simulink library "etherlab_lib"  (Simulink 7.4)
settings: Solver=ode45  SolverMode=SingleTasking  StartTime=0.0  StopTime=10.0  RelTol=1e-3
undefined symbols (not defined in the file or in its folder): baumer_ecatencoder, ekxxxx, el1xxx, el2xxx, el320x_1, el331x, el3356, el3403, el37x2, el4xxx, el500x, el5021, El5152, EL51x1, el51xx, el9xxx, ep1xxx, ep2xxx, ep41xx_1, ep8309, murr_dio
(part 2 of 4)

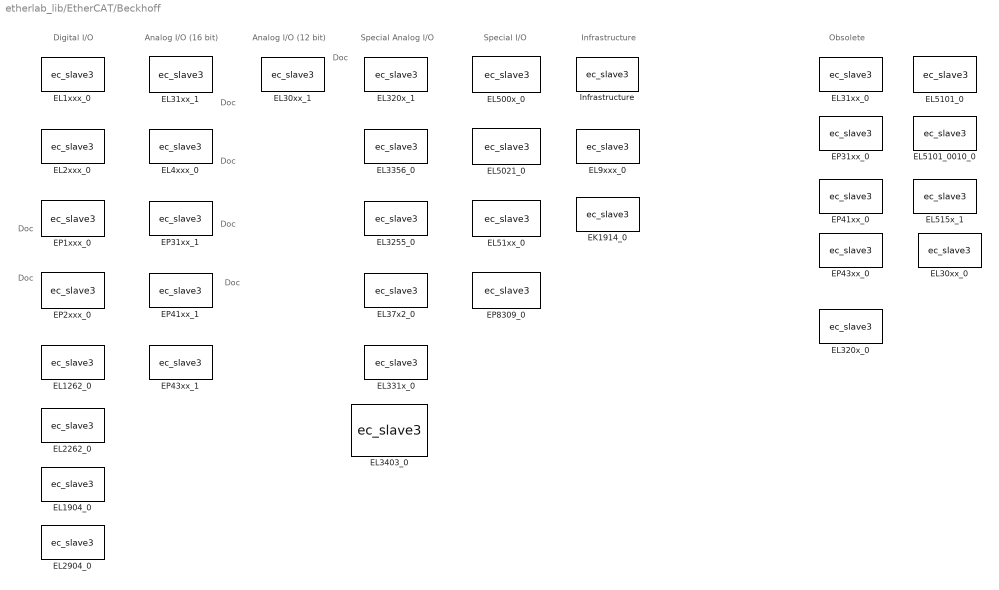
== system etherlab_lib/EtherCAT/Beckhoff ==
  note: Analog I/O (16 bit)
  note: Digital I/O
  note: Analog I/O (12 bit)
  note: Special Analog I/O
  note: Special I/O
  note: Infrastructure
  note: Obsolete
  note: Doc
  note: Doc
  note: Doc
  note: Doc
  note: Doc
  note: Doc
  note: Doc
  EK1914_0 : S-Function  FunctionName=ec_slave3  Parameters=Address,rv.SlaveConfig,rv.PortConfig,debug,tsample  SFunctionModules='ecrt_support'  EnableBusSupport=off  mask(EK1904){master=0, index=1, model=EK1914, stdio=on, safeio=off, tsample=-1, revision=, debug=}
      mask prompts: index "Slave Index"; model "Device Model"; stdio "Standard IO"; safeio "Safe IO"; tsample "Sample Time (-1 for inherited)"
      mask help: Beckhoff EtherCAT SAFE digital input/output coupler
      mask init:
      | Address = EtherCATSlave.formatAddress(master,index,tsample);
      | 
      | rv = ek1914(stdio, safeio);
      | 
      | text = sprintf('%s\\nM:%i Idx:%s', model, master, mat2str(index));
      | if numel(rv.PortConfig.input) > 1 || numel(rv.PortConfig.output) > 1
      |     EtherCATSlave.setPortNames(...
      |         {rv.PortConfig.input.portname},...
      |         {rv.PortConfig.output.portname});
      | 
      |     set_param(gcbh,'AttributesFormatString',text);
      | else
      |     set_param(gcbh,'AttributesFormatString','');
      |     set_param(gcbh,'MaskDisplay', strcat('disp(''',text,''')'));
      | end
      settings: AttributesFormatString=EK1914\nM:0 Idx:1
      mask Help: web(etherlab_help_path('ek1914.html'), '-helpbrowser');
      mask StyleString: edit,edit,popup(EK1914),checkbox,checkbox,edit,edit,edit
      mask Display:
      | port_label('input', 1, 'FSoE')
      | port_label('input', 2, 'StdOut')
      | port_label('output', 1, 'FSoE')
      | port_label('output', 2, 'StdIn')
  EL1262_0 : S-Function  FunctionName=ec_slave3  Parameters=Address,rv.SlaveConfig,rv.PortConfig,debug,tsample  SFunctionModules='ecrt_support'  EnableBusSupport=off  mask(EL1262){master=0, index=1, model=EL1262, one_ch=on, tsample=0, debug=0, revision=, dc_mode=10, dc_assign_activate=hex2dec('730'), dc_cycle0=0, dc_cycle0_factor=-10, dc_shift0=-10000, dc_shift0_factor=1, dc_shift0_input=off, dc_cycle1=0, dc_cycle1_factor=-1, dc_shift1=0, dc_shift1_factor=0}
      mask prompts: index "Slave Index"; model "Device Model"; one_ch "1 Ch. only"; tsample "Sample Time"; dc_mode "Mode/Oversampling"; dc_assign_activate "Assign Activate"; dc_cycle0 "Cycle Time Sync 0 [ns]"; dc_cycle0_factor "Factor"; dc_shift0 "Shift Time Sync0 [ns]"; dc_shift0_factor "Factor"; dc_shift0_input "Shift Time0 Input"; dc_cycle1 "Cycle Time Sync1 [ns]"; dc_cycle1_factor "Factor"; dc_shift1 "Shift Time Sync1 [ns]"; dc_shift1_factor "Factor"
      mask help: Beckhoff oversampling digital input
      mask init:
      | Address = EtherCATSlave.formatAddress(master,index,tsample);
      | 
      | rv = el1262(model).configure(one_ch,...
      |     [dc_mode, dc_assign_activate, ...
      |     dc_cycle0, dc_cycle0_factor,...
      |     dc_shift0, dc_shift0_factor, dc_shift0_input,...
      |     dc_cycle1, dc_cycle1_factor,...
      |     dc_shift1, dc_shift1_factor]);
      mask Help: web(etherlab_help_path('el1262.html'), '-helpbrowser');
      mask StyleString: edit,edit,popup(EL1262|EL1262-0050),checkbox,edit,edit,edit,popup(1|2|3|4|5|8|10|16|20|25|32|40|50|100|200|400|1000|Custom),edit,min,max,min,max,checkbox,min,max,min,max
      mask CallbackString: ||el1262().updateRevision()|||||EtherCATSlave.updateCustomDCEnable();||||||||||
      mask TabNameString: Main,Main,Main,Main,Main,Main,Main,Oversampling/DC,Oversampling/DC,Oversampling/DC,Oversampling/DC,Oversampling/DC,Oversampling/DC,Oversampling/DC,Oversampling/DC,Oversampling/DC,Oversampling/DC,Oversampling/DC
      mask Display: fprintf('%s\nM:%i Idx:%s', model, master, mat2str(index))
  EL1904_0 : S-Function  FunctionName=ec_slave3  Parameters=Address,rv.SlaveConfig,rv.PortConfig,debug,tsample  SFunctionModules='ecrt_support'  EnableBusSupport=off  mask(EL1904){master=0, index=1, model=EL1904, safein=off, tsample=-1, revision=, debug=}
      mask prompts: index "Slave Index"; model "Device Model"; safein "Safe inputs"; tsample "Sample Time (-1 for inherited)"
      mask help: Beckhoff EtherCAT SAFE digital input
      mask init:
      | Address = EtherCATSlave.formatAddress(master,index,tsample);
      | 
      | rv = el1904(safein);
      mask Help: web(etherlab_help_path('el1904.html'), '-helpbrowser');
      mask StyleString: edit,edit,popup(EL1904),checkbox,edit,edit,edit
      mask Display: fprintf('%s\nM:%i Idx:%s', model, master, mat2str(index))
  EL1xxx_0 : S-Function  LoadFcn=el1xxx().checkModelName  FunctionName=ec_slave3  Parameters=Address,rv.SlaveConfig,rv.PortConfig,debug,tsample  SFunctionModules='ecrt_support'  EnableBusSupport=off  mask(EL1xxx){master=0, index=1, model=EL1004, revision=, vector=on, tsample=0, debug=0}
      mask prompts: index "Slave Index"; model "Device Model"; vector "Vector Outputs"; tsample "Sample Time"; debug "Debug Level"
      mask help: Beckhoff EtherCAT Digital Input
      mask init:
      | Address = EtherCATSlave.formatAddress(master,index,tsample);
      | 
      | rv = el1xxx(model).configure(vector);
      mask Help: web(etherlab_help_path('el1xxx.html'), '-helpbrowser');
      mask StyleString: edit,edit,popup(EL1002|EL1004|EL1004-0010|EL1008|EL1012|EL1014|EL1014-0010|EL1018|EL1024|EL1034|EL1084|EL1088|EL1094|EL1098|EL1104|EL1114|EL1124|EL1134|EL1144|EL1202|EL1702|EL1702-0020|EL1712|EL1712-0020|EL1722|EL1804|EL1808|EL1809|EL1814|EL1819|EL1862|EL1862-0010|EL1872|EL1889),edit,checkbox,edit,edit
      mask CallbackString: ||el1xxx().updateRevision()||||
      mask Display: fprintf('%s\nM:%i Idx:%s', model, master, mat2str(index))
  EL2262_0 : S-Function  FunctionName=ec_slave3  Parameters=Address,rv.SlaveConfig,rv.PortConfig,debug,tsample  SFunctionModules='ecrt_support'  EnableBusSupport=off  mask(EL2262){master=0, index=1, model=EL2262, one_ch=on, tsample=0, debug=0, revision=, dc_mode=10, dc_assign_activate=hex2dec('730'), dc_cycle0=0, dc_cycle0_factor=-10, dc_shift0=-10000, dc_shift0_factor=1, dc_shift0_input=off, dc_cycle1=0, dc_cycle1_factor=-1, dc_shift1=0, dc_shift1_factor=0}
      mask prompts: index "Slave Index"; model "Device Model"; one_ch "1 Ch. only"; tsample "Sample Time"; dc_mode "Mode/Oversampling"; dc_assign_activate "Assign Activate"; dc_cycle0 "Cycle Time Sync 0 [ns]"; dc_cycle0_factor "Factor"; dc_shift0 "Shift Time Sync0 [ns]"; dc_shift0_factor "Factor"; dc_shift0_input "Shift Time0 Input"; dc_cycle1 "Cycle Time Sync1 [ns]"; dc_cycle1_factor "Factor"; dc_shift1 "Shift Time Sync1 [ns]"; dc_shift1_factor "Factor"
      mask help: Beckhoff oversampling digital output
      mask init:
      | Address = EtherCATSlave.formatAddress(master,index,tsample);
      | 
      | rv = el2262(model).configure(one_ch,...
      |     [dc_mode, dc_assign_activate, ...
      |     dc_cycle0, dc_cycle0_factor,...
      |     dc_shift0, dc_shift0_factor, dc_shift0_input,...
      |     dc_cycle1, dc_cycle1_factor,...
      |     dc_shift1, dc_shift1_factor]);
      mask Help: web(etherlab_help_path('el2262.html'), '-helpbrowser');
      mask StyleString: edit,edit,popup(EL2262),checkbox,edit,edit,edit,popup(1|2|3|4|5|8|10|16|20|25|32|40|50|100|200|400|1000|Custom),edit,min,max,min,max,checkbox,min,max,min,max
      mask CallbackString: ||el2262().updateRevision()|||||EtherCATSlave.updateCustomDCEnable();||||||||||
      mask TabNameString: Main,Main,Main,Main,Main,Main,Main,Oversampling/DC,Oversampling/DC,Oversampling/DC,Oversampling/DC,Oversampling/DC,Oversampling/DC,Oversampling/DC,Oversampling/DC,Oversampling/DC,Oversampling/DC,Oversampling/DC
      mask Display: fprintf('%s\nM:%i Idx:%s', model, master, mat2str(index))
  EL2904_0 : S-Function  FunctionName=ec_slave3  Parameters=Address,rv.SlaveConfig,rv.PortConfig,debug,tsample  SFunctionModules='ecrt_support'  EnableBusSupport=off  mask(EL2904){master=0, index=1, model=EL2904, safeout=off, tsample=-1, revision=, debug=}
      mask prompts: index "Slave Index"; model "Device Model"; safeout "Safe outputs"; tsample "Sample Time (-1 for inherited)"
      mask help: Beckhoff EtherCAT SAFE digital output
      mask init:
      | Address = EtherCATSlave.formatAddress(master,index,tsample);
      | 
      | rv = el2904(safeout);
      mask Help: web(etherlab_help_path('el2904.html'), '-helpbrowser');
      mask StyleString: edit,edit,popup(EL2904),checkbox,edit,edit,edit
      mask Display: fprintf('%s\nM:%i Idx:%s', model, master, mat2str(index))
  EL2xxx_0 : S-Function  LoadFcn=el2xxx().checkModelName  FunctionName=ec_slave3  Parameters=Address,rv.SlaveConfig,rv.PortConfig,debug,tsample  SFunctionModules='ecrt_support'  EnableBusSupport=off  mask(EL2xxx){master=0, index=1, model=EL2004, revision=, vector=on, diag=off, tsample=-1, debug=0}
      mask prompts: index "Slave Index"; model "Device Model"; vector "Vector Inputs"; diag "Diag Port"; tsample "Sample Time (-1 for inherited)"
      mask help: Beckhoff EtherCAT Digital Output
      mask init:
      | Address = EtherCATSlave.formatAddress(master,index,tsample);
      | 
      | rv = el2xxx(model).configure(vector,diag);
      mask Help: web(etherlab_help_path('el2xxx.html'), '-helpbrowser')
      mask StyleString: edit,edit,popup(EL2002|EL2004|EL2008|EL2022|EL2024|EL2024-0010|EL2032|EL2034|EL2042|EL2084|EL2088|EL2124|EL2202|EL2202-0100|EL2602|EL2612|EL2622|EL2624|EL2652|EL2712|EL2722|EL2722-0010|EL2732|EL2784|EL2788|EL2794|EL2798|EL2808|EL2809|EL2828|EL2872|EL2872-0010|EL2889|EL2004-0000-0000|EL2032-0000-0000|EM2042),edit,checkbox,checkbox,edit,edit
      mask CallbackString: ||el2xxx().modelChanged()|||||
      mask Display: fprintf('%s\nM:%i Idx:%s', model, master, mat2str(index))
  EL30xx_0 : S-Function  LoadFcn=|  FunctionName=ec_slave3  Parameters=Address,rv.SlaveConfig,rv.PortConfig,debug,tsample  SFunctionModules='ecrt_support'  EnableBusSupport=off  mask(EL30xx){master=0, index=1, model=EL3002, vector=on, raw=off, scale=, offset=, tau=, tsample=0, debug=0}
      | el30xx('check')
      | if ~strcmp(bdroot(gcb),'etherlab_lib')
      |   disp([gcb ' is obsolete. Please replace'])
      | end
      mask prompts: index "Slave Index"; model "Device Model"; vector "Vector Output"; raw "Raw Bits"; scale "Output Scale"; offset "Output Offset"; tau "LPF Time Constant (sec)"; tsample "Sample Time"
      mask help: Beckhoff 1,2,4,8-Channel 16-Bit Analog Input
      mask init:
      | Address = EtherCATSlave.formatAddress(master,index,tsample);
      | 
      | el30xx('set');
      | 
      | rv = get_param(gcbh, 'UserData');
      mask StyleString: edit,edit,popup(EL3001|EL3002|EL3004|EL3008|EL3011|EL3012|EL3014|EL3021|EL3022|EL3024|EL3041|EL3042|EL3044|EL3048|EL3051|EL3052|EL3054|EL3058|EL3061|EL3062|EL3062-0030|EL3064|EL3068),checkbox,checkbox,edit,edit,edit,edit,edit
      mask CallbackString: ||el30xx('set');|el30xx('set');||||||
      mask Display:
      | fprintf('%s\n%s AIn\nM:%i Idx:%s', ...
      |     model, rv.SlaveConfig.function, master, mat2str(index))
  EL30xx_1 : S-Function  LoadFcn=|  FunctionName=ec_slave3  Parameters=Address,rv.SlaveConfig,rv.PortConfig,debug,tsample  SFunctionModules='ecrt_support'  EnableBusSupport=off  mask(EL30xx){master=0, index=1, model=EL3002, revision=, vector=on, status=off, gain=[], offset=[], tau=[], tsample=0, debug=0, omega=, filter=Off, opmode=FreeRun, fastop=off}
      | el30xx_1().checkModelName()
      | EtherCATSlave.checkFilter()
      mask prompts: index "Slave Index"; model "Device Model"; vector "Vector Output"; status "Status Output"; gain "Output Scale"; offset "Output Offset"; tau "LPF time constant (s)"; tsample "Sample Time"; omega "deprecated"; opmode "Synchronization Mode (1C33:01.0)"; fastop "FastOp Mode (1C33:01.15)"
      mask help: Beckhoff 1,2,4,8-Channel 16-Bit Analog Input
      mask init:
      | Address = EtherCATSlave.formatAddress(master,index,tsample);
      | 
      | rv = el30xx_1(model).configure(status,vector,...
      |     EtherCATSlave.configureScale(2^15,gain,offset,tau),...
      |     [filter,opmode,fastop]);
      | 
      | if vector
      |     set_param(gcb,'AttributesFormatString','');
      | 
      |     set_param(gcb,'MaskDisplay',...
      |         sprintf('disp(''%s %s\\nM:%i Idx:%s'')',...
      |         model,rv.function,master,mat2str(index)))
      | else
      |     EtherCATSlave.setPortNames({},...
      |         {rv.PortConfig.output.portname})
      |     
      |     set_param(gcb,'AttributesFormatString',...
      |         sprintf('%s %s\nM:%i Idx:%s',...
      |         model,rv.function,master,mat2str(index)))
      | end
      mask StyleString: edit,edit,popup(EL3001|EL3002|EL3004|EL3008|EL3011|EL3012|EL3014|EL3021|EL3022|EL3024|EL3041|EL3042|EL3042-0017|EL3044|EL3048|EL3051|EL3052|EL3054|EL3058|EL3061|EL3062|EL3062-0015|EL3062-0030|EL3064|EL3068|EL3001-0000-0018|EL3002-0000-0018|EL3004-0000-0018|EL3008-0000-0018|EL3011-0000-0016|EL3012-0000-0016|EL3014-0000-0016|EL3021-0000-0016|EL3022-0000-0016|EL3024-0000-0016|EL3041-0000-0017|EL3042-0000-0017|EL3044-0000-0017|EL3048-0000-0017|EL3051-0000-0017|EL3052-0000-0017|EL3054-0000-0017|EL3058-0000-0017|EL3061-0000-0017|EL3062-0000-0017|EL3062-0030-0017|EL3064-0000-0017|EL3068-0000-0017),edit,checkbox,checkbox,edit,edit,edit,edit,edit,edit,popup(Off|50Hz FIR|60Hz FIR|IIR 1|IIR 2|IIR 3|IIR 4|IIR 5|IIR 6|IIR 7|IIR 8),popup(FreeRun|FrameTriggered SM2),checkbox
      mask CallbackString: ||el30xx_1().updateRevision()||||||||||el30xx_1.updateFilter||
      mask TabNameString: Main,Main,Main,Main,Main,Main,Main,Main,Main,Main,Main,Main,Filter,Filter,Filter
      mask Display: disp('EL3002 +-10V\nM:0 Idx:1')
  EL31xx_0 : S-Function  LoadFcn=|  FunctionName=ec_slave3  Parameters=Address,rv.SlaveConfig,rv.PortConfig,debug,tsample  SFunctionModules='ecrt_support'  EnableBusSupport=off  mask(EL31xx){master=0, index=1, model=EL3102, dc=DC-Synchron, vector=on, raw=off, scale=, offset=, tau=, tsample=0, debug=0}
      | el31xx('check')
      | if ~strcmp(bdroot(gcb),'etherlab_lib')
      |   disp([gcb ' is obsolete. Please replace'])
      | end
      mask prompts: index "Slave Index"; model "Device Model"; dc "Distributed Clock"; vector "Vector Output"; raw "Raw output"; scale "Output Scale"; offset "Output Offset"; tau "LPF Time Constant (sec)"; tsample "Sample Time"
      mask help:
      | Beckhoff 2,4,8-Channel 16-Bit Analog Input with Distributed Clocks
      |
      | Status output is not supported
      mask init:
      | Address = EtherCATSlave.formatAddress(master,index,tsample);
      | 
      | el31xx('set');  % Report errors
      | 
      | rv = get_param(gcb,'UserData');
      mask Help:
      | This block generically implements the EtherCAT 16-Bit Analog Input Terminal for various models.
      | <p/>
      | The following Terminals are supported:
      | <center>
      | <table width="80%">
      | <tr><td>EL3102,4,8</td><td>-10..10V Voltage Input</td></tr>
      | <tr><td>EL3112,4   </td><td>0..20mA Current Input</td></tr>
      | <tr><td>EL3122,4   </td><td>4..20mA Current Input</td></tr>
      | <tr><td>EL3142,4,8</td><td>0..20mA Current Input</td></tr>
      | <tr><td>EL3152,4,8</td><td>4..20mA Current Input</td></tr>
      | <tr><td>EL3162,4,8</td><td>0..10V Voltage Input</td></tr>
      | </table>
      | </center>
      | <p/>
      | Choose and set the following options:
      | <h4>Master:</h4>
      | Set the EtherCAT Master of this terminal.
      | 
      | <h4>Slave Index:</h4>
      | Set the EtherCAT slave index. Following address formats are allowed:
      | <ol>
      | <li> Absolute addressing: a scalar number <<b><tt>n</tt></b>> representing the (zero based) absolute position in the bus.
      | <li> SSId addressing: the Secondary Slave (or 'Alias') Addressing has the form <<b><tt>[alias position]</tt></b>> where <b><tt>alias</tt></b> is the Secondary Slave Id of the EtherCAT slave and <b><tt>position</tt></b> is the offset after the slave with the given <b><tt>alias</tt></b>. The SSId has to be preprogrammed into the slave with other service tools (see 'ethercat alias --help').
      | </ol>
      | 
      | <h4>Device Model:</h4>
      | Choose the model at the Indexed position of the master.
      | 
      | <h4>Output Type:</h4>
      | <ul>
      | <li>Choose <b>Vector Output</b> to have a single output as a vector
      | with a size corresponding to the channel count of the terminal. This mode also allows a status output port to be displayed. <br/>
      | <li>Choose <b>Separate Outputs</b> to have one output for every channel.
      | </ul>
      | <h4>Output Full Scale</h4>
      | When <b>Output Data Type</b> is set to <b>Double with scale and offset</b>, the block's output value at full scale terminal input can be set here.
      | 
      | <h4>Output Offset</h4>
      | When <b>Output Data Type</b> is set to <b>Double with scale and offset</b>, the blocks output at zero terminal input can be set here. Note that the Full Scale above is also increased by this amount. Note furthermore that this corresponds to the minimum input for terminals such as 4..20mA.
      | 
      | <h4>Output Data Type</h4>
      | Choose the block's output data type for the output signal. Available are:
      | <ul>
      | <li><b><tt>Raw</tt></b> outputting the internal raw value as <tt>int16_T</tt> or <tt>uint16_T</tt> as appropriate
      | <li><b><tt>Double</tt></b> outputting 0..10, -10..10, 0..0.02 and 0.004..0.02 depending on the Model as appropriate
      | <li><b><tt>Double with scale and offset</tt></b>, allowing the output to be scaled with an offset.
      | </ul>
      | 
      | <p>
      | Choosing <b>Status Output</b> provides a port of type <tt>uint8_T</tt> where the status is presented. This is only enabled when <b>Vector Output</b> is selected. Terminal input over- and underrange can be detected using this output. See the terminal's documentation.
      | 
      | <h4>Output Filter</h4>
      | When not in <b>Raw</b> mode, the <b>Output Filter</b> checkbox becomes available, allowing the use of an internal low pass filter. Enter the <b>LPF Time Constant</b> for the filter in the field below.
      | <br>For continuous sample time systems (0 in Sample Time), the filter is also continuous. Discrete samples systems (Sample Time > 0) uses an equivalent discrete low pass filter with a similar time constant.
      | 
      | <p>
      | Set the <b>Sample Time</b> for the block. <tt>0</tt> is continuous sample time (runs at the model's base rate). Setting <tt>-1</tt> will try to set the time using back propagation.
      mask StyleString: edit,edit,popup(EL3101|EL3102|EL3104|EL3111|EL3112|EL3114|EL3121|EL3122|EL3124|EL3141|EL3142|EL3142-010|EL3144|EL3151|EL3152|EL3154|EL3161|EL3162|EL3164),popup(Free Run|DC-Synchron|DC-Synchron (input based)),checkbox,checkbox,edit,edit,edit,edit,edit
      mask CallbackString: ||el31xx('set')|el31xx('set')|el31xx('set')||||||
      mask Display:
      | fprintf('%s\n%s AIn\nM:%i Idx:%s', ...
      |     model, rv.SlaveConfig.function, master, mat2str(index))
  EL31xx_1 : S-Function  LoadFcn=|  FunctionName=ec_slave3  Parameters=Address,rv.SlaveConfig,rv.PortConfig,debug,tsample  SFunctionModules='ecrt_support'  EnableBusSupport=off  mask(EL31xx){master=0, index=1, model=EL3102, revision=, vector=on, status=off, filter=Off, gain=[], offset=[], tau=[], tsample=0, debug=0, omega=, dc_mode=Free Run/SM-Synchron, dc_assign_activate=hex2dec('700'), dc_cycle0=[], dc_cycle0_factor=[], dc_shift0=[], dc_shift0_factor=[], dc_shift0_input=off, dc_cycle1=[], dc_cycle1_factor=[], dc_shift1=[], dc_shift1_factor=[]}
      | el31xx_1().checkModelName()
      | EtherCATSlave.checkFilter()
      mask prompts: index "Slave Index"; model "Device Model"; vector "Vector Output"; status "Status output"; gain "Output Gain"; offset "Output Offset"; tau "LPF time constant (s)"; tsample "Sample Time"; omega "deprecated"; dc_mode "Mode"; dc_assign_activate "Assign Activate"; dc_cycle0 "Cycle Time Sync 0"; dc_cycle0_factor "Factor"; dc_shift0 "Shift Time Sync0"; dc_shift0_factor "Factor"; dc_shift0_input "Shift Time0 Input"; dc_cycle1 "Cycle Time Sync1"; dc_cycle1_factor "Factor"; dc_shift1 "Shift Time Sync1"; dc_shift1_factor "Factor"
      mask help: Beckhoff 2,4,8-Channel 16-Bit Analog Input with Distributed Clocks
      mask init:
      | Address = EtherCATSlave.formatAddress(master,index,tsample);
      | 
      | rv = el31xx_1(model).configure(status,vector,...
      |     EtherCATSlave.configureScale(2^15,gain,offset,tau),...
      |     [dc_mode, dc_assign_activate, ...
      |      dc_cycle0, dc_cycle0_factor, ...
      |      dc_shift0, dc_shift0_factor, dc_shift0_input, ...
      |      dc_cycle1, dc_cycle1_factor, ...
      |      dc_shift1, dc_shift1_factor], ...
      |      filter);
      |  
      | if vector || model(6) == '1'
      |     set_param(gcb,'AttributesFormatString','');
      | 
      |     set_param(gcb,'MaskDisplay',...
      |         sprintf('disp(''%s\\nM:%i Idx:%s'')',...
      |         model,master,mat2str(index)))
      | else
      |     EtherCATSlave.setPortNames({},...
      |         {rv.PortConfig.output.portname})
      |     
      |     set_param(gcb,'AttributesFormatString',...
      |         sprintf('%s\nM:%i Idx:%s',...
      |         model,master,mat2str(index)))
      | end
      mask Help:
      | This block generically implements the EtherCAT 16-Bit Analog Input Terminal for various models.
      | <p/>
      | The following Terminals are supported:
      | <center>
      | <table width="80%">
      | <tr><td>EL3102,4,8</td><td>-10..10V Voltage Input</td></tr>
      | <tr><td>EL3112,4   </td><td>0..20mA Current Input</td></tr>
      | <tr><td>EL3122,4   </td><td>4..20mA Current Input</td></tr>
      | <tr><td>EL3142,4,8</td><td>0..20mA Current Input</td></tr>
      | <tr><td>EL3152,4,8</td><td>4..20mA Current Input</td></tr>
      | <tr><td>EL3162,4,8</td><td>0..10V Voltage Input</td></tr>
      | </table>
      | </center>
      | <p/>
      | Choose and set the following options:
      | <h4>Master:</h4>
      | Set the EtherCAT Master of this terminal.
      | 
      | <h4>Slave Index:</h4>
      | Set the EtherCAT slave index. Following address formats are allowed:
      | <ol>
      | <li> Absolute addressing: a scalar number <<b><tt>n</tt></b>> representing the (zero based) absolute position in the bus.
      | <li> SSId addressing: the Secondary Slave (or 'Alias') Addressing has the form <<b><tt>[alias position]</tt></b>> where <b><tt>alias</tt></b> is the Secondary Slave Id of the EtherCAT slave and <b><tt>position</tt></b> is the offset after the slave with the given <b><tt>alias</tt></b>. The SSId has to be preprogrammed into the slave with other service tools (see 'ethercat alias --help').
      | </ol>
      | 
      | <h4>Device Model:</h4>
      | Choose the model at the Indexed position of the master.
      | 
      | <h4>Output Type:</h4>
      | <ul>
      | <li>Choose <b>Vector Output</b> to have a single output as a vector
      | with a size corresponding to the channel count of the terminal. This mode also allows a status output port to be displayed. <br/>
      | <li>Choose <b>Separate Outputs</b> to have one output for every channel.
      | </ul>
      | <h4>Output Full Scale</h4>
      | When <b>Output Data Type</b> is set to <b>Double with scale and offset</b>, the block's output value at full scale terminal input can be set here.
      | 
      | <h4>Output Offset</h4>
      | When <b>Output Data Type</b> is set to <b>Double with scale and offset</b>, the blocks output at zero terminal input can be set here. Note that the Full Scale above is also increased by this amount. Note furthermore that this corresponds to the minimum input for terminals such as 4..20mA.
      | 
      | <h4>Output Data Type</h4>
      | Choose the block's output data type for the output signal. Available are:
      | <ul>
      | <li><b><tt>Raw</tt></b> outputting the internal raw value as <tt>int16_T</tt> or <tt>uint16_T</tt> as appropriate
      | <li><b><tt>Double</tt></b> outputting 0..10, -10..10, 0..0.02 and 0.004..0.02 depending on the Model as appropriate
      | <li><b><tt>Double with scale and offset</tt></b>, allowing the output to be scaled with an offset.
      | </ul>
      | 
      | <p>
      | Choosing <b>Status Output</b> provides a port of type <tt>uint8_T</tt> where the status is presented. This is only enabled when <b>Vector Output</b> is selected. Terminal input over- and underrange can be detected using this output. See the terminal's documentation.
      | 
      | <h4>Output Filter</h4>
      | When not in <b>Raw</b> mode, the <b>Output Filter</b> checkbox becomes available, allowing the use of an internal low pass filter. Enter the <b>LPF Time Constant</b> for the filter in the field below.
      | <br>For continuous sample time systems (0 in Sample Time), the filter is also continuous. Discrete samples systems (Sample Time > 0) uses an equivalent discrete low pass filter with a similar time constant.
      | 
      | <p>
      | Set the <b>Sample Time</b> for the block. <tt>0</tt> is continuous sample time (runs at the model's base rate). Setting <tt>-1</tt> will try to set the time using back propagation.
      mask StyleString: edit,edit,popup(EL3101|EL3102|EL3104|EL3111|EL3112|EL3114|EL3121|EL3122|EL3124|EL3141|EL3142|EL3142-0010|EL3144|EL3151|EL3152|EL3154|EL3161|EL3162|EL3164|EL3101-0000-0016|EL3102-0000-0017|EL3104-0000-0016|EL3111-0000-0016|EL3112-0000-0017|EL3114-0000-0017|EL3121-0000-0016|EL3122-0000-0017|EL3124-0000-0016|EL3141-0000-0016|EL3142-0000-0017|EL3142-0010-0017|EL3144-0000-0016|EL3151-0000-0016|EL3152-0000-0017|EL3154-0000-0016|EL3161-0000-0016|EL3162-0000-0017|EL3164-0000-0016),edit,checkbox,checkbox,popup(Off|50Hz FIR|60Hz FIR|IIR 1|IIR 2|IIR 3|IIR 4|IIR 5|IIR 6|IIR 7|IIR 8),edit,edit,edit,edit,edit,edit,popup(Free Run/SM-Synchron|DC-Synchron|DC-Synchron (input based)|Custom),edit,min,max,min,max,checkbox,min,max,min,max
      mask CallbackString: ||el31xx_1().updateRevision()|el31xx_1().updateRevision()||||||||||EtherCATSlave.updateCustomDCEnable()||||||||||
      mask TabNameString: Main,Main,Main,Main,Main,Main,Main,Main,Main,Main,Main,Main,Main,Distributed Clocks,Distributed Clocks,Distributed Clocks,Distributed Clocks,Distributed Clocks,Distributed Clocks,Distributed Clocks,Distributed Clocks,Distributed Clocks,Distributed Clocks,Distributed Clocks
      mask Display: disp('EL3102\nM:0 Idx:1')
  EL320x_0 : S-Function  LoadFcn=|  FunctionName=ec_slave3  Parameters=Address,rv.SlaveConfig,rv.PortConfig,debug,tsample  SFunctionModules='ecrt_support'  EnableBusSupport=off  mask(EL320x){master=0, index=1, model=EL3204, rtd=0, technology=2, filter=50 Hz, vector=on, enable_status=on, tsample=0, debug=0}
      | el320x('check')
      | if ~strcmp(bdroot(gcb),'etherlab_lib')
      |   disp([gcb ' is obsolete. Please replace'])
      | end
      mask prompts: index "Slave Index"; model "Device Model"; rtd "RTD-Element (CoE 80x0:19)"; technology "Connection Technology (CoE 80x0:1A)"; filter "Filter (CoE 8000:15)"; vector "Vector Output"; enable_status "Status Port"; tsample "Sample Time"
      mask help: Beckhoff 1, 2, 4-Channel Input Terminal Pt100 (RTD)
      mask init:
      | Address = EtherCATSlave.formatAddress(master,index,tsample);
      | 
      | SdoConfig = [];
      | 
      | rv = get_param(gcbh,'UserData');
      | 
      | count = numel(rv.SlaveConfig.sm{1}{3});
      | 
      | err = {};
      | if numel(rtd) == 1
      |     rtd = repmat(rtd,1,count);
      | elseif numel(rtd) ~= count
      |     err = {['- Mask option "RTD Element"' ...
      |         ' is not a scalar or vector with ' ...
      |         num2str(count) ' elements']};
      | end
      | 
      | if numel(technology) == 1
      |     technology = repmat(technology,1,count);
      | elseif numel(technology) ~= count
      |     err = horzcat(err, ['- Mask option "Connection Technology"' ...
      |         ' is not a scalar or vector with ' ...
      |         num2str(count) ' elements']);
      | end
      | 
      | if ~isempty(err)
      |     errordlg(err,gcb);
      |     return
      | end
      | 
      | rv.SlaveConfig.sdo = num2cell(vertcat(...
      |     [hex2dec('8000'),6,8,1],...
      |     [hex2dec('8000'),hex2dec('15'),16,filter+1],...
      |     horzcat(repmat(hex2dec('8000') + 16*(0:count-1)',2,1),...
      |             [hex2dec('19')*ones(count,1);hex2dec('1a')*ones(count,1)],...
      |             16*ones(count*2,1),...
      |             vertcat(reshape(rtd,[],1),...
      |                     reshape(technology,[],1)))));
      mask Help: web(etherlab_help_path('el320x.html'), '-helpbrowser');
      mask StyleString: edit,edit,popup(EL3201|EL3201-0010|EL3201-0020|EL3202|EL3202-0010|EL3204),edit,edit,popup(50 Hz|60 Hz|100 Hz|500 Hz|1 kHz|2 kHz|3.75 kHz|7.5 kHz|15 kHz|30 kHz|5 Hz|10 Hz),checkbox,checkbox,edit,edit
      mask CallbackString: ||el320x('set');||||el320x('set');|el320x('set');||
      mask Display: fprintf('%s\nRTD In\n%i Idx:%s', model, master, mat2str(index))
  EL320x_1 : S-Function  LoadFcn=el320x_1().checkModelName()  FunctionName=ec_slave3  Parameters=Address,rv.SlaveConfig,rv.PortConfig,debug,tsample  SFunctionModules='ecrt_support'  EnableBusSupport=off  mask(EL320x){master=0, index=1, model=EL3201, revision=, filter=Off, vector=on, status=off, tsample=0, debug=0, sdo_01=Pt100 -200...850C, sdo_02=2-wire, sdo_03=0, sdo_04=Pt100 -200...850C, sdo_05=2-wire, sdo_06=0, sdo_07=Pt100 -200...850C, sdo_08=2-wire, sdo_09=0, sdo_10=Pt100 -200...850C, sdo_11=2-wire, sdo_12=0, sdo_13=Pt100 -200...850C, sdo_14=2-wire, sdo_15=0, sdo_16=Pt100 -200...850C, sdo_17=2-wire, sdo_18=0, sdo_19=Pt100 -200...850C, sdo_20=2-wire, sdo_21=0, sdo_22=Pt100 -200...850C, sdo_23=2-wire, sdo_24=0}
      mask prompts: index "Slave Index"; model "Device Model"; vector "Vector Output"; status "Status Port"; tsample "Sample Time"; sdo_01 "RTD-Element"; sdo_02 "Technology"; sdo_03 "Wire Calibration (1/32 Ohm)"; sdo_04 "RTD-Element"; sdo_05 "Technology"; sdo_06 "Wire Calibration (1/32 Ohm)"; sdo_07 "RTD-Element"; sdo_08 "Technology"; sdo_09 "Wire Calibration (1/32 Ohm)"; sdo_10 "RTD-Element"; sdo_11 "Technology"; sdo_12 "Wire Calibration (1/32 Ohm)"; sdo_13 "RTD-Element"; sdo_14 "Technology"; sdo_15 "Wire Calibration (1/32 Ohm)"; sdo_16 "RTD-Element"; sdo_17 "Technology"; sdo_18 "Wire Calibration (1/32 Ohm)"; sdo_19 "RTD-Element"; sdo_20 "Technology"; sdo_21 "Wire Calibration (1/32 Ohm)"; sdo_22 "RTD-Element"; sdo_23 "Technology"; sdo_24 "Wire Calibration (1/32 Ohm)"
      mask help: Beckhoff 1, 2, 4-Channel Input Terminal Pt100 (RTD)
      mask init:
      | Address = EtherCATSlave.formatAddress(master,index,tsample);
      | 
      | rv = el320x_1(model).configure(status,vector,filter,...
      |     [sdo_01,sdo_04,sdo_07,sdo_10,sdo_13,sdo_16,sdo_19,sdo_22] - 1,...
      |     [sdo_02,sdo_05,sdo_08,sdo_11,sdo_14,sdo_17,sdo_20,sdo_23] - 1,...
      |     [sdo_03,sdo_06,sdo_09,sdo_12,sdo_15,sdo_18,sdo_21,sdo_24]);
      | 
      | if vector || model(6) == '1'
      |     set_param(gcb,'AttributesFormatString','');
      | 
      |     set_param(gcb,'MaskDisplay',...
      |         sprintf('disp(''%s\\nM:%i Idx:%s'')',...
      |         model,master,mat2str(index)))
      | else
      |     EtherCATSlave.setPortNames({},...
      |         {rv.PortConfig.output.portname})
      |     
      |     set_param(gcb,'AttributesFormatString',...
      |         sprintf('%s\nM:%i Idx:%s',...
      |         model,master,mat2str(index)))
      | end
      mask Help: web(etherlab_help_path('el320x.html'), '-helpbrowser');
      mask StyleString: edit,edit,popup(EL3201|EL3201-0010|EL3201-0020|EL3202|EL3202-0010|EL3202-0020|EL3204|EL3204-0200|EL3208|EL3214),edit,popup(Off|50 Hz|60 Hz|100 Hz|500 Hz|1 kHz|2 kHz|3.75 kHz|7.5 kHz|15 kHz|30 kHz|5 Hz|10 Hz),checkbox,checkbox,edit,edit,popup(Pt100 -200...850C|Ni100 -60...250C|Pt1000 -200...850C|Pt500 -200...850C|Pt200 -200...850C|Ni1000 -60...250C|Ni1000 100C: 1500 Ohm (-30...60C)|Ni120 -60...320C|1/16 Ohm (10 .. 4095 Ohm) |1/64 Ohm (10 .. 1047 Ohm) |KT100/110/130/210/230 KTY10/11/13/16/19  |KTY81/82-110/120/150 (-50...150C)|KTY81-121|KTY81-122|KTY81-151|KTY81-152|KTY81/82-210/220/250|KTY81-221|KTY81-222|KTY81-251|KTY81-252|KTY83-110/120/150 (-50...175C)|KTY83-121|KTY83-122|KTY83-151|KTY83-152|KTY84-130/150 (-40...300C)|KTY84-151|KTY21/23-6 (-50...150C)|KTY1x-5|KTY1x-7|KTY21/23-5|KTY21/23-7),popup(2-wire|3-wire|4-wire|Not connected),edit,popup(Pt100 -200...850C|Ni100 -60...250C|Pt1000 -200...850C|Pt500 -200...850C|Pt200 -200...850C|Ni1000 -60...250C|Ni1000 100C: 1500 Ohm (-30...60C)|Ni120 -60...320C|1/16 Ohm (10 .. 4095 Ohm) |1/64 Ohm (10 .. 1047 Ohm) |KT100/110/130/210/230 KTY10/11/13/16/19  |KTY81/82-110/120/150 (-50...150C)|KTY81-121|KTY81-122|KTY81-151|KTY81-152|KTY81/82-210/220/250|KTY81-221|KTY81-222|KTY81-251|KTY81-252|KTY83-110/120/150 (-50...175C)|KTY83-121|KTY83-122|KTY83-151|KTY83-152|KTY84-130/150 (-40...300C)|KTY84-151|KTY21/23-6 (-50...150C)|KTY1x-5|KTY1x-7|KTY21/23-5|KTY21/23-7),popup(2-wire|3-wire|4-wire|Not connected),edit,popup(Pt100 -200...850C|Ni100 -60...250C|Pt1000 -200...850C|Pt500 -200...850C|Pt200 -200...850C|Ni1000 -60...250C|Ni1000 100C: 1500 Ohm (-30...60C)|Ni120 -60...320C|1/16 Ohm (10 .. 4095 Ohm) |1/64 Ohm (10 .. 1047 Ohm) |KT100/110/130/210/230 KTY10/11/13/16/19  |KTY81/82-110/120/150 (-50...150C)|KTY81-121|KTY81-122|KTY81-151|KTY81-152|KTY81/82-210/220/250|KTY81-221|KTY81-222|KTY81-251|KTY81-252|KTY83-110/120/150 (-50...175C)|KTY83-121|KTY83-122|KTY83-151|KTY83-152|KTY84-130/150 (-40...300C)|KTY84-151|KTY21/23-6 (-50...150C)|KTY1x-5|KTY1x-7|KTY21/23-5|KTY21/23-7),popup(2-wire|3-wire|4-wire|Not connected),edit,popup(Pt100 -200...850C|Ni100 -60...250C|Pt1000 -200...850C|Pt500 -200...850C|Pt200 -200...850C|Ni1000 -60...250C|Ni1000 100C: 1500 Ohm (-30...60C)|Ni120 -60...320C|1/16 Ohm (10 .. 4095 Ohm) |1/64 Ohm (10 .. 1047 Ohm) |KT100/110/130/210/230 KTY10/11/13/16/19  |KTY81/82-110/120/150 (-50...150C)|KTY81-121|KTY81-122|KTY81-151|KTY81-152|KTY81/82-210/220/250|KTY81-221|KTY81-222|KTY81-251|KTY81-252|KTY83-110/120/150 (-50...175C)|KTY83-121|KTY83-122|KTY83-151|KTY83-152|KTY84-130/150 (-40...300C)|KTY84-151|KTY21/23-6 (-50...150C)|KTY1x-5|KTY1x-7|KTY21/23-5|KTY21/23-7),popup(2-wire|3-wire|4-wire|Not connected),edit,popup(Pt100 -200...850C|Ni100 -60...250C|Pt1000 -200...850C|Pt500 -200...850C|Pt200 -200...850C|Ni1000 -60...250C|Ni1000 100C: 1500 Ohm (-30...60C)|Ni120 -60...320C|1/16 Ohm (10 .. 4095 Ohm) |1/64 Ohm (10 .. 1047 Ohm) |KT100/110/130/210/230 KTY10/11/13/16/19  |KTY81/82-110/120/150 (-50...150C)|KTY81-121|KTY81-122|KTY81-151|KTY81-152|KTY81/82-210/220/250|KTY81-221|KTY81-222|KTY81-251|KTY81-252|KTY83-110/120/150 (-50...175C)|KTY83-121|KTY83-122|KTY83-151|KTY83-152|KTY84-130/150 (-40...300C)|KTY84-151|KTY21/23-6 (-50...150C)|KTY1x-5|KTY1x-7|KTY21/23-5|KTY21/23-7),popup(2-wire|3-wire|4-wire|Not connected),edit,popup(Pt100 -200...850C|Ni100 -60...250C|Pt1000 -200...850C|Pt500 -200...850C|Pt200 -200...850C|Ni1000 -60...250C|Ni1000 100C: 1500 Ohm (-30...60C)|Ni120 -60...320C|1/16 Ohm (10 .. 4095 Ohm) |1/64 Ohm (10 .. 1047 Ohm) |KT100/110/130/210/230 KTY10/11/13/16/19  |KTY81/82-110/120/150 (-50...150C)|KTY81-121|KTY81-122|KTY81-151|KTY81-152|KTY81/82-210/220/250|KTY81-221|KTY81-222|KTY81-251|KTY81-252|KTY83-110/120/150 (-50...175C)|KTY83-121|KTY83-122|KTY83-151|KTY83-152|KTY84-130/150 (-40...300C)|KTY84-151|KTY21/23-6 (-50...150C)|KTY1x-5|KTY1x-7|KTY21/23-5|KTY21/23-7),popup(2-wire|3-wire|4-wire|Not connected),edit,popup(Pt100 -200...850C|Ni100 -60...250C|Pt1000 -200...850C|Pt500 -200...850C|Pt200 -200...850C|Ni1000 -60...250C|Ni1000 100C: 1500 Ohm (-30...60C)|Ni120 -60...320C|1/16 Ohm (10 .. 4095 Ohm) |1/64 Ohm (10 .. 1047 Ohm) |KT100/110/130/210/230 KTY10/11/13/16/19  |KTY81/82-110/120/150 (-50...150C)|KTY81-121|KTY81-122|KTY81-151|KTY81-152|KTY81/82-210/220/250|KTY81-221|KTY81-222|KTY81-251|KTY81-252|KTY83-110/120/150 (-50...175C)|KTY83-121|KTY83-122|KTY83-151|KTY83-152|KTY84-130/150 (-40...300C)|KTY84-151|KTY21/23-6 (-50...150C)|KTY1x-5|KTY1x-7|KTY21/23-5|KTY21/23-7),popup(2-wire|3-wire|4-wire|Not connected),edit,popup(Pt100 -200...850C|Ni100 -60...250C|Pt1000 -200...850C|Pt500 -200...850C|Pt200 -200...850C|Ni1000 -60...250C|Ni1000 100C: 1500 Ohm (-30...60C)|Ni120 -60...320C|1/16 Ohm (10 .. 4095 Ohm) |1/64 Ohm (10 .. 1047 Ohm) |KT100/110/130/210/230 KTY10/11/13/16/19  |KTY81/82-110/120/150 (-50...150C)|KTY81-121|KTY81-122|KTY81-151|KTY81-152|KTY81/82-210/220/250|KTY81-221|KTY81-222|KTY81-251|KTY81-252|KTY83-110/120/150 (-50...175C)|KTY83-121|KTY83-122|KTY83-151|KTY83-152|KTY84-130/150 (-40...300C)|KTY84-151|KTY21/23-6 (-50...150C)|KTY1x-5|KTY1x-7|KTY21/23-5|KTY21/23-7),popup(2-wire|3-wire|4-wire|Not connected),edit
      mask CallbackString: ||el320x_1.modelChanged()||||||||||||||||||||||||||||||
      mask TabNameString: Main,Main,Main,Main,Main,Main,Main,Main,Main,Sensor 1,Sensor 1,Sensor 1,Sensor 2,Sensor 2,Sensor 2,Sensor 3,Sensor 3,Sensor 3,Sensor 4,Sensor 4,Sensor 4,Sensor 5,Sensor 5,Sensor 5,Sensor 6,Sensor 6,Sensor 6,Sensor 7,Sensor 7,Sensor 7,Sensor 8,Sensor 8,Sensor 8
      mask Display: disp('EL3201\nM:0 Idx:1')
  EL3255_0 : S-Function  LoadFcn=|  FunctionName=ec_slave3  Parameters=Address,rv.SlaveConfig,rv.PortConfig,debug,tsample  SFunctionModules='ecrt_support'  EnableBusSupport=off  mask(EL3255){master=0, index=1, model=EL3255, revision=, channels=1, vector=off, gain=[], offset=[], tau=[], tsample=0, debug=0, omega=, dc_mode=Free Run/SM-Synchron, dc_assign_activate=hex2dec('700'), dc_cycle0=[], dc_cycle0_factor=[], dc_shift0=[], dc_shift0_factor=[], dc_shift0_input=off, dc_cycle1=[], dc_cycle1_factor=[], dc_shift1=[], dc_shift1_factor=[], sdo_01=off, sdo_02=50 Hz, sdo_03=Off (up to 10 kOhm), sdo_04=Off (up to 10 kOhm), sdo_05=Off (up to 10 kOhm), sdo_06=Off (up to 10 kOhm), sdo_07=Off (up to 10 kOhm)}
      | el3255().checkModelName()
      | EtherCATSlave.checkFilter
      mask prompts: index "Slave Index"; model "Device Model"; channels "Active Channels"; vector "Vector Outputs"; tau "LPF time constant (s)"; tsample "Sample Time"; debug "Debug Level"; omega "deprecated"; dc_mode "Distributed Clock"; dc_assign_activate "Assign Activate"; dc_cycle0 "Cycle Time Sync 0"; dc_cycle0_factor "Factor"; dc_shift0 "Shift Time Sync0"; dc_shift0_factor "Factor"; dc_shift0_input "Shift Time0 Input"; dc_cycle1 "Cycle Time Sync1"; dc_cycle1_factor "Factor"; dc_shift1 "Shift Time Sync1"; dc_shift1_factor "Factor"; sdo_01 "Enable Filter (#x8000:06)"; sdo_02 "Filter settings (#x8000:15)"; sdo_03 "Load resistance 1"; sdo_04 "Load resistance 2"; sdo_05 "Load resistance 3"; sdo_06 "Load resistance 4"; sdo_07 "Load resistance 5"
      mask help: Beckhoff EtherCAT 5Ch. potentiometer measurement with sensor supply
      mask init:
      | Address = EtherCATSlave.formatAddress(master,index,tsample);
      | 
      | rv = el3255(model).configure(channels,vector,...
      |     [dc_mode, dc_assign_activate, ...
      |     dc_cycle0, dc_cycle0_factor,...
      |     dc_shift0, dc_shift0_factor, dc_shift0_input,...
      |     dc_cycle1, dc_cycle1_factor,...
      |     dc_shift1, dc_shift1_factor], ...
      |     EtherCATSlave.configureScale(2^15,gain,offset,tau),...
      |     [sdo_01, ...
      |      [sdo_02, sdo_03, sdo_04, sdo_05, sdo_06, sdo_07]-1]);
      mask Help: web(etherlab_help_path('el3255.html'), '-helpbrowser');
      mask StyleString: edit,edit,popup(EL3255),edit,popup(1|1..2|1..3|1..4|1..5),checkbox,edit,edit,edit,edit,edit,edit,popup(Free Run/SM-Synchron|DC-Synchron|DC-Synchron (input based)|Custom),edit,min,max,min,max,checkbox,min,max,min,max,checkbox,popup(50 Hz|60 Hz|100 Hz|500 Hz|1 kHz|2 kHz|3.75 kHz|7.5 kHz|15 kHz|30 kHz|5 Hz|10 Hz),popup(Off (up to 10 kOhm)|25 kOhm|50 kOhm),popup(Off (up to 10 kOhm)|25 kOhm|50 kOhm),popup(Off (up to 10 kOhm)|25 kOhm|50 kOhm),popup(Off (up to 10 kOhm)|25 kOhm|50 kOhm),popup(Off (up to 10 kOhm)|25 kOhm|50 kOhm)
      mask CallbackString: ||el3255().updateRevision()||||||||||EtherCATSlave.updateCustomDCEnable();|||||||||||||||||
      mask TabNameString: Main,Main,Main,Main,Main,Main,Main,Main,Main,Main,Main,Main,Distributed Clocks,Distributed Clocks,Distributed Clocks,Distributed Clocks,Distributed Clocks,Distributed Clocks,Distributed Clocks,Distributed Clocks,Distributed Clocks,Distributed Clocks,Distributed Clocks,CoE,CoE,CoE,CoE,CoE,CoE,CoE
      mask Display: fprintf('%s\nM:%i Idx:%s', model, master, mat2str(index))
  EL331x_0 : S-Function  LoadFcn=el331x().checkModelName  FunctionName=ec_slave3  Parameters=Address,rv.SlaveConfig,rv.PortConfig,debug,tsample  SFunctionModules='ecrt_support'  EnableBusSupport=off  mask(EL331x){master=0, index=1, model=EL3314, revision=, vector=on, status=off, tsample=0, debug=0, sdo_8000_02=0.1, sdo_8000_0C=Internal, sdo_8000_15=50 Hz, sdo_8000_19=0: Type K, sdo_8000_1A=Inactive, sdo_8010_02=0.1, sdo_8010_0C=Internal, sdo_8010_15=50 Hz, sdo_8010_19=0: Type K, sdo_8010_1A=Inactive, sdo_8020_02=0.1, sdo_8020_0C=Internal, sdo_8020_15=50 Hz, sdo_8020_19=0: Type K, sdo_8020_1A=Inactive, sdo_8030_02=0.1, sdo_8030_0C=Internal, sdo_8030_15=50 Hz, sdo_8030_19=0: Type K, sdo_8030_1A=Inactive, sdo_8040_02=0.1, sdo_8040_0C=Internal, sdo_8040_15=50 Hz, sdo_8040_19=0: Type K, sdo_8040_1A=Inactive, sdo_8050_02=0.1, sdo_8050_0C=Internal, sdo_8050_15=50 Hz, sdo_8050_19=0: Type K, sdo_8050_1A=Inactive, sdo_8060_02=0.1, sdo_8060_0C=Internal, sdo_8060_15=50 Hz, sdo_8060_19=0: Type K, sdo_8060_1A=Inactive, sdo_8070_02=0.1, sdo_8070_0C=Internal, sdo_8070_15=50 Hz, sdo_8070_19=0: Type K, sdo_8070_1A=Inactive}
      mask prompts: index "Slave Index"; model "Device Model"; vector "Vector Outputs"; status "Status Output"; tsample "Sample Time"; sdo_8000_02 "Resolution (#x8000:02)"; sdo_8000_0C "Coldjunction Compensation (#x8000:0C)"; sdo_8000_15 "Filter settings (#x8000:15)"; sdo_8000_19 "TC Element (#x8000:19)"; sdo_8000_1A "MC Filter (#x8000:1A)"; sdo_8010_02 "Resolution (#x8010:02)"; sdo_8010_0C "Coldjunction Compensation (#x8010:0C)"; sdo_8010_15 "Filter settings (#x8010:15)"; sdo_8010_19 "TC Element (#x8010:19)"; sdo_8010_1A "MC Filter (#x8010:1A)"; sdo_8020_02 "Resolution (#x8020:02)"; sdo_8020_0C "Coldjunction Compensation (#x8020:0C)"; sdo_8020_15 "Filter settings (#x8020:15)"; sdo_8020_19 "TC Element (#x8020:19)"; sdo_8020_1A "MC Filter (#x8020:1A)"; sdo_8030_02 "Resolution (#x8030:02)"; sdo_8030_0C "Coldjunction Compensation (#x8030:0C)"; sdo_8030_15 "Filter settings (#x8030:15)"; sdo_8030_19 "TC Element (#x8030:19)"; sdo_8030_1A "MC Filter (#x8030:1A)"; sdo_8040_02 "Resolution (#x8040:02)"; sdo_8040_0C "Coldjunction Compensation (#x8040:0C)"; sdo_8040_15 "Filter settings (#x8040:15)"; sdo_8040_19 "TC Element (#x8040:19)"; sdo_8040_1A "MC Filter (#x8040:1A)"; sdo_8050_02 "Resolution (#x8050:02)"; sdo_8050_0C "Coldjunction Compensation (#x8050:0C)"; sdo_8050_15 "Filter settings (#x8050:15)"; sdo_8050_19 "TC Element (#x8050:19)"; sdo_8050_1A "MC Filter (#x8050:1A)"; sdo_8060_02 "Resolution (#x8060:02)"; sdo_8060_0C "Coldjunction Compensation (#x8060:0C)"; sdo_8060_15 "Filter settings (#x8060:15)"; sdo_8060_19 "TC Element (#x8060:19)"; sdo_8060_1A "MC Filter (#x8060:1A)"; sdo_8070_02 "Resolution (#x8070:02)"; sdo_8070_0C "Coldjunction Compensation (#x8070:0C)"; sdo_8070_15 "Filter settings (#x8070:15)"; sdo_8070_19 "TC Element (#x8070:19)"; sdo_8070_1A "MC Filter (#x8070:1A)"
      mask help: Beckhoff thermocouple input slave terminal
      mask init:
      | Address = EtherCATSlave.formatAddress(master,index,tsample);
      | 
      | rv = el331x(model).configure(vector,status,...
      |     [sdo_8000_02,sdo_8000_0C,sdo_8000_15,sdo_8000_19,sdo_8000_1A;
      |      sdo_8010_02,sdo_8010_0C,sdo_8010_15,sdo_8010_19,sdo_8010_1A;
      |      sdo_8020_02,sdo_8020_0C,sdo_8020_15,sdo_8020_19,sdo_8020_1A;
      |      sdo_8030_02,sdo_8030_0C,sdo_8030_15,sdo_8030_19,sdo_8030_1A;
      |      sdo_8040_02,sdo_8040_0C,sdo_8040_15,sdo_8040_19,sdo_8040_1A;
      |      sdo_8050_02,sdo_8050_0C,sdo_8050_15,sdo_8050_19,sdo_8050_1A;
      |      sdo_8060_02,sdo_8060_0C,sdo_8060_15,sdo_8060_19,sdo_8060_1A;
      |      sdo_8070_02,sdo_8070_0C,sdo_8070_15,sdo_8070_19,sdo_8070_1A]);
      mask Help: web(etherlab_help_path('el331x.html'), '-helpbrowser');
      mask StyleString: edit,edit,popup(EL3311|EL3312|EL3314|EL3314-0010|EL3318),edit,checkbox,checkbox,edit,edit,popup(0.1|0.01|0.001 (EL3314-0010 only)),popup(Internal|None|External Process Data),popup(50 Hz|60 Hz|100 Hz|500 Hz|1 kHz|2 kHz|3.75 kHz|7.5 kHz|15 kHz|30 kHz|5 Hz|10 Hz),popup(0: Type K|1: Type J|2: Type L|3: Type E|4: Type T|5: Type N|6: Type U|7: Type B|8: Type R|9: Type S|10: Type C|100: 30mV|101: 60mV|102: 75mV|104: 78mV),popup(Inactive|IIR 1|IIR 2|IIR 3|IIR 4|FIR 1|FIR 8|FIR 16|FIR 32),popup(0.1|0.01|0.001 (EL3314-0010 only)),popup(Internal|None|External Process Data),popup(50 Hz|60 Hz|100 Hz|500 Hz|1 kHz|2 kHz|3.75 kHz|7.5 kHz|15 kHz|30 kHz|5 Hz|10 Hz),popup(0: Type K|1: Type J|2: Type L|3: Type E|4: Type T|5: Type N|6: Type U|7: Type B|8: Type R|9: Type S|10: Type C|100: 30mV|101: 60mV|102: 75mV|104: 78mV),popup(Inactive|IIR 1|IIR 2|IIR 3|IIR 4|FIR 1|FIR 8|FIR 16|FIR 32),popup(0.1|0.01|0.001 (EL3314-0010 only)),popup(Internal|None|External Process Data),popup(50 Hz|60 Hz|100 Hz|500 Hz|1 kHz|2 kHz|3.75 kHz|7.5 kHz|15 kHz|30 kHz|5 Hz|10 Hz),popup(0: Type K|1: Type J|2: Type L|3: Type E|4: Type T|5: Type N|6: Type U|7: Type B|8: Type R|9: Type S|10: Type C|100: 30mV|101: 60mV|102: 75mV|104: 78mV),popup(Inactive|IIR 1|IIR 2|IIR 3|IIR 4|FIR 1|FIR 8|FIR 16|FIR 32),popup(0.1|0.01|0.001 (EL3314-0010 only)),popup(Internal|None|External Process Data),popup(50 Hz|60 Hz|100 Hz|500 Hz|1 kHz|2 kHz|3.75 kHz|7.5 kHz|15 kHz|30 kHz|5 Hz|10 Hz),popup(0: Type K|1: Type J|2: Type L|3: Type E|4: Type T|5: Type N|6: Type U|7: Type B|8: Type R|9: Type S|10: Type C|100: 30mV|101: 60mV|102: 75mV|104: 78mV),popup(Inactive|IIR 1|IIR 2|IIR 3|IIR 4|FIR 1|FIR 8|FIR 16|FIR 32),popup(0.1|0.01|0.001 (EL3314-0010 only)),popup(Internal|None|External Process Data),popup(50 Hz|60 Hz|100 Hz|500 Hz|1 kHz|2 kHz|3.75 kHz|7.5 kHz|15 kHz|30 kHz|5 Hz|10 Hz),popup(0: Type K|1: Type J|2: Type L|3: Type E|4: Type T|5: Type N|6: Type U|7: Type B|8: Type R|9: Type S|10: Type C|100: 30mV|101: 60mV|102: 75mV|104: 78mV),popup(Inactive|IIR 1|IIR 2|IIR 3|IIR 4|FIR 1|FIR 8|FIR 16|FIR 32),popup(0.1|0.01|0.001 (EL3314-0010 only)),popup(Internal|None|External Process Data),popup(50 Hz|60 Hz|100 Hz|500 Hz|1 kHz|2 kHz|3.75 kHz|7.5 kHz|15 kHz|30 kHz|5 Hz|10 Hz),popup(0: Type K|1: Type J|2: Type L|3: Type E|4: Type T|5: Type N|6: Type U|7: Type B|8: Type R|9: Type S|10: Type C|100: 30mV|101: 60mV|102: 75mV|104: 78mV),popup(Inactive|IIR 1|IIR 2|IIR 3|IIR 4|FIR 1|FIR 8|FIR 16|FIR 32),popup(0.1|0.01|0.001 (EL3314-0010 only)),popup(Internal|None|External Process Data),popup(50 Hz|60 Hz|100 Hz|500 Hz|1 kHz|2 kHz|3.75 kHz|7.5 kHz|15 kHz|30 kHz|5 Hz|10 Hz),popup(0: Type K|1: Type J|2: Type L|3: Type E|4: Type T|5: Type N|6: Type U|7: Type B|8: Type R|9: Type S|10: Type C|100: 30mV|101: 60mV|102: 75mV|104: 78mV),popup(Inactive|IIR 1|IIR 2|IIR 3|IIR 4|FIR 1|FIR 8|FIR 16|FIR 32),popup(0.1|0.01|0.001 (EL3314-0010 only)),popup(Internal|None|External Process Data),popup(50 Hz|60 Hz|100 Hz|500 Hz|1 kHz|2 kHz|3.75 kHz|7.5 kHz|15 kHz|30 kHz|5 Hz|10 Hz),popup(0: Type K|1: Type J|2: Type L|3: Type E|4: Type T|5: Type N|6: Type U|7: Type B|8: Type R|9: Type S|10: Type C|100: 30mV|101: 60mV|102: 75mV|104: 78mV),popup(Inactive|IIR 1|IIR 2|IIR 3|IIR 4|FIR 1|FIR 8|FIR 16|FIR 32)
      mask CallbackString: ||el331x.modelChanged||el331x.updateVector|||||||||||||||||||||||||||||||||||||||||||
      mask TabNameString: Main,Main,Main,Main,Main,Main,Main,Main,Ch.1,Ch.1,Ch.1,Ch.1,Ch.1,Ch.2,Ch.2,Ch.2,Ch.2,Ch.2,Ch.3,Ch.3,Ch.3,Ch.3,Ch.3,Ch.4,Ch.4,Ch.4,Ch.4,Ch.4,Ch.5,Ch.5,Ch.5,Ch.5,Ch.5,Ch.6,Ch.6,Ch.6,Ch.6,Ch.6,Ch.7,Ch.7,Ch.7,Ch.7,Ch.7,Ch.8,Ch.8,Ch.8,Ch.8,Ch.8
      mask Display: fprintf('%s\nM:%i Idx:%s', model, master, mat2str(index))
  EL3356_0 : S-Function  LoadFcn=el3356().checkModelName()  FunctionName=ec_slave3  Parameters=Address,rv.SlaveConfig,rv.PortConfig,debug,tsample  SFunctionModules='ecrt_support'  EnableBusSupport=off  mask(EL3356){master=0, index=1, model=EL3356, revision=, adc=off, range=[], scale=[], offset=[], tau=[], tsample=-1, debug=0, omega=, dc_mode=SM-Synchron, dc_assign_activate=hex2dec('320'), dc_cycle0=0, dc_cycle0_factor=1, dc_shift0=0, dc_shift0_factor=0, dc_shift0_input=off, dc_cycle1=0, dc_cycle1_factor=1, dc_shift1=0, dc_shift1_factor=0, sdo_01=off, sdo_02=off, sdo_03=on, sdo_04=on, sdo_05=off, sdo_06=FIR 50 Hz, sdo_07=FIR 50 Hz, sdo_08=10, sdo_09=hex2dec(num2hex(single(20))), sdo_10=1000, sdo_11=5, sdo_12=1800, sdo_13=10, sdo_14=off, sdo_15=50 Hz FIR, sdo_16=off, sdo_17=50 Hz FIR}
      mask prompts: index "Slave Index"; model "Device Model"; adc "2 ch ADC only"; range "RMB Range [mV/V]"; scale "Output Scale"; offset "Output Offset"; tau "LPF time constant (s)"; tsample "Sample Time"; omega "deprecated"; dc_mode "Mode"; dc_assign_activate "Assign Activate"; dc_cycle0 "Cycle Time Sync 0"; dc_cycle0_factor "Factor"; dc_shift0 "Shift Time Sync0"; dc_shift0_factor "Factor"; dc_shift0_input "Shift Time0 Input"; dc_cycle1 "Cycle Time Sync1"; dc_cycle1_factor "Factor"; dc_shift1 "Shift Time Sync1"; dc_shift1_factor "Factor"; sdo_01 "Mode 0 Enable Filter (#x8000:01)"; sdo_02 "Mode 1 Enable Filter (#x8000:02)"; sdo_03 "Mode 0 Enable Averager (#x8000:03)"; sdo_04 "Mode 1 Enable Averager (#x8000:04)"; sdo_05 "Symmetric Reference Potential (#x8000:05)"; sdo_06 "Mode 0 Filter (#x8000:11)"; sdo_07 "Mode 1 Filter (#x8000:12)"; sdo_08 "Dynamic filter change time [0.01s] (#x8000:13)"; sdo_09 "Dynamic filter delta (#x8000:14) (binary value)"; sdo_10 "Steady state window (#x8000:29)"; sdo_11 "Steady state tolerance (#x8000:2a)"; sdo_12 "Calibration interval [100ms] (#x8000:31)"; sdo_13 "Test interval (#x8000:32)"; sdo_14 "Enable ch. 1 filter (#x8010:06)"; sdo_15 "Ch.1 filter settings (#x8010:15)"; sdo_16 "Enable ch.2 filter (#x8020:06)"; sdo_17 "Ch.2 filter settings (#x8020:15)"
      mask help: Beckhoff DMS Input with Distributed Clocks
      mask init:
      | Address = EtherCATSlave.formatAddress(master,index,tsample);
      | 
      | rv = el3356(model).configure(adc,range,...
      |     [dc_mode, dc_assign_activate, ...
      |     dc_cycle0, dc_cycle0_factor,...
      |     dc_shift0, dc_shift0_factor, dc_shift0_input,...
      |     dc_cycle1, dc_cycle1_factor,...
      |     dc_shift1, dc_shift1_factor], ...
      |     EtherCATSlave.configureScale(2^31,scale,offset,tau),...
      |     [sdo_01,   sdo_02,   sdo_03, sdo_04, sdo_05, ...
      |      sdo_06-1, sdo_07-1, sdo_08, sdo_09, sdo_10, ...
      |      sdo_11,   sdo_12,   sdo_13, ...
      |      sdo_14,   sdo_15-1, ...
      |      sdo_16,   sdo_17-1]);
      |  
      | EtherCATSlave.setPortNames(...
      |     {rv.PortConfig.input.portname},...
      |     {rv.PortConfig.output.portname});
      | 
      | set_param(gcb,'AttributesFormatString',...
      |     sprintf('%s\nM:%i Idx:%s',...
      |             model,master,mat2str(index)))
      settings: AttributesFormatString=|
      | EL3356
      | M:0 Idx:1
      mask Help: web(etherlab_help_path('el3356.html'), '-helpbrowser');
      mask StyleString: edit,edit,popup(EL3356|EL3356-0010),edit,checkbox,edit,edit,edit,edit,edit,edit,edit,popup(SM-Synchron|DC-Synchron|DC-Synchron (input based)|Custom),edit,min,max,min,max,checkbox,min,max,min,max,checkbox,checkbox,checkbox,checkbox,checkbox,popup(FIR 50 Hz|FIR 60 Hz|IIR 1|IIR 2|IIR 3|IIR 4|IIR 5|IIR 6|IIR 7|IIR 8|Dynamic IIR),popup(FIR 50 Hz|FIR 60 Hz|IIR 1|IIR 2|IIR 3|IIR 4|IIR 5|IIR 6|IIR 7|IIR 8|Dynamic IIR),edit,edit,edit,edit,edit,edit,checkbox,popup(50 Hz FIR|60 Hz FIR|IIR 1|IIR 2|IIR 3|IIR 4|IIR 5|IIR 6|IIR 7|IIR 8),checkbox,popup(50 Hz FIR|60 Hz FIR|IIR 1|IIR 2|IIR 3|IIR 4|IIR 5|IIR 6|IIR 7|IIR 8)
      mask CallbackString: ||el3356.modelChanged()||||||||||EtherCATSlave.updateCustomDCEnable();|||||||||||||||||||||||||||
      mask TabNameString: Main,Main,Main,Main,Main,Main,Main,Main,Main,Main,Main,Main,Distributed Clocks,Distributed Clocks,Distributed Clocks,Distributed Clocks,Distributed Clocks,Distributed Clocks,Distributed Clocks,Distributed Clocks,Distributed Clocks,Distributed Clocks,Distributed Clocks,CoE #x8000,CoE #x8000,CoE #x8000,CoE #x8000,CoE #x8000,CoE #x8000,CoE #x8000,CoE #x8000,CoE #x8000,CoE #x8000,CoE #x8000,CoE #x8000,CoE #x8000,CoE #x80x0,CoE #x80x0,CoE #x80x0,CoE #x80x0
      mask Display:
      | port_label('input', 1, 'Ctrl')
      | port_label('output', 1, 'RMB')
      | port_label('output', 2, 'Status')
  EL3403_0 : S-Function  LoadFcn=el3403().checkModelName()  FunctionName=ec_slave3  Parameters=Address,rv.SlaveConfig,rv.PortConfig,debug,tsample  SFunctionModules='ecrt_support'  EnableBusSupport=off  mask(EL3403){master=0, index=1, model=EL3403, variant=off, current=1, voltage=1, tsample=-1, revision=[223031378 1441792], debug=0, freq=Phase L1, ref=Phase L1, zerocross=5, cycle=10}
      mask prompts: index "Slave Index"; model "Device Model"; variant "Variants"; current "Current Transformation Ratio 1:"; voltage "Voltage Transformation Ratio 1:"; tsample "Sample Time (-1 inherited)"; freq "Frequency channel (F800:05)"; ref "Reference channel (F800:0E)"; zerocross "Zero cross timeout (F800:21)"; cycle "Line cycle (F800:22)"
      mask help: Beckhoff 3-phase power measurement terminal
      mask init:
      | Address = EtherCATSlave.formatAddress(master,index,tsample);
      | 
      | rv = el3403(model).configure(variant,current,voltage,...
      |     [freq-1, ref-1, zerocross, cycle]);
      | 
      | EtherCATSlave.setPortNames(...
      |     {rv.PortConfig.input.portname},...
      |     {rv.PortConfig.output.portname});
      | 
      | set_param(gcb,'AttributesFormatString',...
      |     sprintf('%s\nM:%i Idx:%s',...
      |             model,master,mat2str(index)))
      settings: AttributesFormatString=|
      | EL3403
      | M:0 Idx:1
      mask Help: web(etherlab_help_path('el3403.html'), '-helpbrowser');
      mask StyleString: edit,edit,popup(EL3403|EL3403-0010|EL3403-0026|EL3403-0100|EL3403-0111|EL3403-0126),checkbox,edit,edit,edit,edit,edit,popup(Phase L1|Phase L2|Phase L3),popup(Phase L1|Phase L2|Phase L3),edit,edit
      mask TabNameString: Main,Main,Main,Main,Main,Main,Main,Main,Main,Settings,Settings,Settings,Settings
      mask Display:
      | port_label('output', 1, 'Current')
      | port_label('output', 2, 'Voltage')
      | port_label('output', 3, 'Power')
      | port_label('output', 4, 'Zero Crossing Fail')
      | port_label('output', 5, 'Seq. Fail')
  EL37x2_0 : S-Function  LoadFcn=el37x2().checkModelName()  FunctionName=ec_slave3  Parameters=Address,rv.SlaveConfig,rv.PortConfig,debug,tsample  SFunctionModules='ecrt_support'  EnableBusSupport=off  mask(EL37x2){master=0, index=1, model=EL3702, revision=, one_ch=off, scale=[], offset=[], tsample=0, debug=0, dc_mode=10, dc_assign_activate=hex2dec('730'), dc_cycle0=0, dc_cycle0_factor=-10     % 10-times OS, dc_shift0=-10000, dc_shift0_factor=1, dc_shift0_input=off, dc_cycle1=0, dc_cycle1_factor=-1, dc_shift1=0, dc_shift1_factor=0}
      mask prompts: index "Slave Index"; model "Device Model"; one_ch "1 Ch. only"; scale "Output Scale"; offset "Output Offset"; tsample "Sample Time"; dc_mode "Mode/Oversampling"; dc_assign_activate "Assign Activate"; dc_cycle0 "Cycle Time Sync 0 [ns]"; dc_cycle0_factor "Factor"; dc_shift0 "Shift Time Sync0 [ns]"; dc_shift0_factor "Factor"; dc_shift0_input "Shift Time0 Input"; dc_cycle1 "Cycle Time Sync1 [ns]"; dc_cycle1_factor "Factor"; dc_shift1 "Shift Time Sync1 [ns]"; dc_shift1_factor "Factor"
      mask help: Beckhoff oversampling analog input
      mask init:
      | Address = EtherCATSlave.formatAddress(master,index,tsample);
      | 
      | rv = el37x2(model).configure(one_ch,...
      |     [dc_mode, dc_assign_activate, ...
      |     dc_cycle0, dc_cycle0_factor,...
      |     dc_shift0, dc_shift0_factor, dc_shift0_input,...
      |     dc_cycle1, dc_cycle1_factor,...
      |     dc_shift1, dc_shift1_factor], ...
      |     EtherCATSlave.configureScale(2^15,scale,offset));
      mask Help: web(etherlab_help_path('el37x2.html'), '-helpbrowser');
      mask StyleString: edit,edit,popup(EL3702|EL3742),edit,checkbox,edit,edit,edit,edit,popup(1|2|3|4|5|8|10|16|20|25|32|40|50|100|Custom),edit,min,max,min,max,checkbox,min,max,min,max
      mask CallbackString: ||el37x2().updateRevision()|||||||EtherCATSlave.updateCustomDCEnable();||||||||||
      mask TabNameString: Main,Main,Main,Main,Main,Main,Main,Main,Main,Oversampling/DC,Oversampling/DC,Oversampling/DC,Oversampling/DC,Oversampling/DC,Oversampling/DC,Oversampling/DC,Oversampling/DC,Oversampling/DC,Oversampling/DC,Oversampling/DC
      mask Display: fprintf('%s\nM:%i Idx:%s', model, master, mat2str(index))
  EL4xxx_0 : S-Function  LoadFcn=el4xxx().checkModelName()  FunctionName=ec_slave3  Parameters=Address,rv.SlaveConfig,rv.PortConfig,debug,tsample  SFunctionModules='ecrt_support'  EnableBusSupport=off  mask(EL4xxx){master=0, index=1, model=EL4002, revision=, vector=on, scale=[], tsample=-1, debug=0, dc_mode=Free Run, dc_assign_activate=hex2dec('700'), dc_cycle0=0, dc_cycle0_factor=1, dc_shift0=0, dc_shift0_factor=0, dc_shift0_input=off, dc_cycle1=0, dc_cycle1_factor=1, dc_shift1=10000, dc_shift1_factor=0}
      mask prompts: index "Slave Index"; model "Device Model"; vector "Vector Input"; scale "Input Scale (empty for none)"; tsample "Sample Time (-1 for inherited)"; dc_mode "Distributed Clocks"; dc_assign_activate "Assign Activate"; dc_cycle0 "Cycle Time Sync 0"; dc_cycle0_factor "Factor"; dc_shift0 "Shift Time Sync0"; dc_shift0_factor "Factor"; dc_shift0_input "Shift Time0 Input"; dc_cycle1 "Cycle Time Sync1"; dc_cycle1_factor "Factor"; dc_shift1 "Shift Time Sync1"; dc_shift1_factor "Factor"
      mask help: Beckhoff Analog Output
      mask init:
      | Address = EtherCATSlave.formatAddress(master,index,tsample);
      | 
      | rv = el4xxx(model).configure(vector,...
      |     EtherCATSlave.configureScale(2^15,scale),...
      |     [dc_mode, dc_assign_activate,...
      |      dc_cycle0, dc_cycle0_factor,...
      |      dc_shift0, dc_shift0_factor, dc_shift0_input,...
      |      dc_cycle1, dc_cycle1_factor,...
      |      dc_shift1, dc_shift1_factor]);
      mask Help:
      | This block generically implements the EtherCAT 16-Bit Analog Input Terminal for various models.
      | <p/>
      | The block input is generally a <tt>double</tt> from the range 0..1 for unipolar terminals and -1..1 for bipolar terminals, where 1 is the highest possible output of the terminal.
      | <p/>
      | Exceeding the input range simply saturates the terminal's output.
      | <p/>
      | The following Terminals are supported:
      | <center>
      | <table width="80%">
      | <tr><td>EL4008</td><td>0..10V Voltage Output</td></tr>
      | <tr><td>EL4028</td><td>4..20 mA Current Output</td></tr>
      | <tr><td>EL4034</td><td>-10..10V Voltage Output</td></tr>
      | <tr><td>EL4102</td><td>0..10V Voltage Output</td></tr>
      | <tr><td>EL4112</td><td>0..20mA Current Output</td></tr>
      | <tr><td>EL4122</td><td>4..20mA Current Output</td></tr>
      | <tr><td>EL4132</td><td>-10..10V Voltage Output</td></tr>
      | </table>
      | </center>
      | <p/>
      | Choose and set the following options:
      | <h4>Master:</h4>
      | Set the EtherCAT Master of this terminal.
      | 
      | <h4>Slave Index:</h4>
      | Set the EtherCAT slave index. Following address formats are allowed:
      | <ol>
      | <li> Absolute addressing: a scalar number <<b><tt>n</tt></b>> representing the (zero based) absolute position in the bus.
      | <li> SSId addressing: the Secondary Slave (or 'Alias') Addressing has the form <<b><tt>[alias position]</tt></b>> where <b><tt>alias</tt></b> is the Secondary Slave Id of the EtherCAT slave and <b><tt>position</tt></b> is the offset after the slave with the given <b><tt>alias</tt></b>. The SSId has to be preprogrammed into the slave with other service tools (see 'ethercat alias --help').
      | </ol>
      | 
      | <h4>Device Model:</h4>
      | Choose the device at the Indexed position of the master.
      | 
      | <h4>Input Type:</h4>
      | <ul>
      | <li>Choose <b>Vector Input</b> to have a single input as a vector
      | with a size corresponding to the channel count of the terminal. This mode also allows a control input and a status output port to be displayed.
      | <li>Choose <b>Separate Inputs</b> to have one input for every channel.
      | </ul>
      | 
      | <p>
      | Choosing <b>Status Output</b> provides a port of type <tt>uint8_T</tt> where the status is presented. This is only enabled when <b>Vector Output</b> is selected. Note: at the time of writing (1.2.2006) the terminals do not have a status output, and hence this option is disabled!
      | 
      | <p>
      | All input signals are multiplied with the factor <b>Input Scale</b>.
      | 
      | <p>
      | Set the <b>Sample Time</b> for the block. <tt>0</tt> is continuous sample time (runs at the model's base rate). Setting <tt>-1</tt> will try to set the time using back propagation.
      mask StyleString: edit,edit,popup(EL4001|EL4002|EL4004|EL4008|EL4011|EL4012|EL4014|EL4018|EL4021|EL4022|EL4024|EL4028|EL4031|EL4032|EL4034|EL4038|EL4102|EL4104|EL4112|EL4112-0010|EL4114|EL4122|EL4124|EL4132|EL4134|EL4001-0000-0016|EL4002-0000-0018|EL4002-0000-0016|EL4004-0000-0018|EL4004-0000-0016|EL4008-0000-0018|EL4008-0000-0016|EL4011-0000-0018|EL4011-0000-0016|EL4012-0000-0018|EL4012-0000-0016|EL4014-0000-0018|EL4014-0000-0016|EL4018-0000-0018|EL4018-0000-0016|EL4021-0000-0018|EL4021-0000-0016|EL4022-0000-0018|EL4022-0000-0016|EL4024-0000-0018|EL4024-0000-0016|EL4028-0000-0018|EL4028-0000-0016|EL4031-0000-0018|EL4031-0000-0016|EL4032-0000-0018|EL4032-0000-0016|EL4034-0000-0018|EL4034-0000-0016|EL4038-0000-0018|EL4038-0000-0016),edit,checkbox,edit,edit,edit,popup(Free Run|DC-Synchron|Custom),edit,min,max,min,max,checkbox,min,max,min,max
      mask CallbackString: ||el4xxx().updateRevision()||||||EtherCATSlave.updateCustomDCEnable()||||||||||
      mask TabNameString: Main,Main,Main,Main,Main,Main,Main,Main,Distributed Clocks,Distributed Clocks,Distributed Clocks,Distributed Clocks,Distributed Clocks,Distributed Clocks,Distributed Clocks,Distributed Clocks,Distributed Clocks,Distributed Clocks,Distributed Clocks
      mask Display:
      | fprintf('%s\n%s AIn\nM:%i Idx:%s', ...
      |     model, rv.function, master, mat2str(index))
  EL500x_0 : S-Function  LoadFcn=el500x().checkModelName()  FunctionName=ec_slave3  Parameters=Address,rv.SlaveConfig,rv.PortConfig,debug,tsample  SFunctionModules='ecrt_support'  EnableBusSupport=off  mask(EL500x){master=0, index=1, model=EL5001, revision=, pdo_x1A02=off, tsample=0, debug=0, dc_mode=FreeRun/SM-Synchron, dc_assign_activate=hex2dec('700')    % '120' for EL5001-0011, dc_cycle0=0, dc_cycle0_factor=1, dc_shift0=0, dc_shift0_factor=0, dc_shift0_input=off, dc_cycle1=0, dc_cycle1_factor=1, dc_shift1=15000, dc_shift1_factor=0, sdo_01=off, sdo_02=off, sdo_03=off, sdo_04=off, sdo_05=off, sdo_06=Gray, sdo_07=500k, sdo_08=Multiturn (25 bits), sdo_09=25, sdo_10=24, sdo_11=0, sdo_12=off, sdo_13=off, sdo_14=off, sdo_15=off, sdo_16=Gray, sdo_17=500k, sdo_18=Multiturn (25 bits), sdo_19=25, sdo_20=24, sdo_21=0}
      mask prompts: index "Slave Index"; model "Device Model"; pdo_x1A02 "Timestamp (PDO #x1a02)"; tsample "Sample Time"; dc_mode "DC Mode"; dc_assign_activate "Assign Activate"; dc_cycle0 "Cycle Time Sync 0 [ns]"; dc_cycle0_factor "Factor"; dc_shift0 "Shift Time Sync0 [ns]"; dc_shift0_factor "Factor"; dc_shift0_input "Shift Time0 Input"; dc_cycle1 "Cycle Time Sync1 [ns]"; dc_cycle1_factor "Factor"; dc_shift1 "Shift Time Sync1 [ns]"; dc_shift1_factor "Factor"; sdo_01 "8000:01 - Disable frame error"; sdo_02 "8000:02 - Enable power failure bit"; sdo_03 "8000:03 - Enable inhibit time"; sdo_04 "8000:04 - Enable test mode"; sdo_05 "8000:05 - Check SSI-frame size"; sdo_06 "8000:06 - SSI-coding"; sdo_07 "8000:09 - SSI-baudrate"; sdo_08 "8000:0F - SSI-frame type"; sdo_09 "8000:11 - SSI-frame size"; sdo_10 "8000:12 - SSI-data length"; sdo_11 "8000:13 - Min Inhibit Time [us]"; sdo_12 "8010:01 - Disable frame error"; sdo_13 "8010:02 - Enable power failure bit"; sdo_14 "8010:03 - Enable inhibit time"; sdo_15 "8010:04 - Enable test mode"; sdo_16 "8010:06 - SSI-coding"; sdo_17 "8010:09 - SSI-baudrate"; sdo_18 "8010:0F - SSI-frame type"; sdo_19 "8010:11 - SSI-frame size"; sdo_20 "8010:12 - SSI-data length"; sdo_21 "8010:13 - Min Inhibit Time [us]"
      mask help: Beckhoff EtherCAT SSI Input
      mask init:
      | Address = EtherCATSlave.formatAddress(master,index,tsample);
      | 
      | rv = el500x(model).configure(pdo_x1A02, ...
      |     [  sdo_01,   sdo_02, sdo_03,   sdo_04,   sdo_05, sdo_06-1,...
      |      sdo_07-1, sdo_08-1, sdo_09,   sdo_10,   sdo_11,   sdo_12,...
      |      sdo_13-1,   sdo_14, sdo_15, sdo_16-1, sdo_17-1, sdo_18-1,...
      |        sdo_19,   sdo_20, sdo_21],...
      |     [dc_mode, dc_assign_activate, ...
      |      dc_cycle0, dc_cycle0_factor,...
      |      dc_shift0, dc_shift0_factor, dc_shift0_input,...
      |      dc_cycle1, dc_cycle1_factor,...
      |      dc_shift1, dc_shift1_factor]);
      | 
      | if numel(rv.PortConfig.output) > 2
      |     EtherCATSlave.setPortNames({},...
      |         {rv.PortConfig.output.portname});
      |     
      |     set_param(gcb,'AttributesFormatString',...
      |         sprintf('%s\nM:%i Idx:%s',...
      |         model,master,mat2str(index)))
      | else
      |     set_param(gcb,'AttributesFormatString','');
      | 
      |     set_param(gcb,'MaskDisplay',...
      |         sprintf('disp(''%s\\nM:%i Idx:%s'')',...
      |         model,master,mat2str(index)))
      | end
      mask Help: web(etherlab_help_path('el500x.html'), '-helpbrowser');
      mask StyleString: edit,edit,popup(EL5001|EL5001-0011|EL5002),edit,checkbox,edit,edit,popup(FreeRun/SM-Synchron|DC-Synchron|DC-Synchron (input based)|DC-Latch active (only for EL5001-001x)|Custom),edit,min,max,min,max,checkbox,min,max,min,max,checkbox,checkbox,checkbox,checkbox,checkbox,popup(Binary|Gray),popup(1250k|1000k|500k|250k|125k),popup(Multiturn (25 bits)|Singleturn (13 bits)|Variable (set size in Frame Size)),edit,edit,edit,checkbox,checkbox,checkbox,checkbox,popup(Binary|Gray),popup(1250k|1000k|500k|250k|125k),popup(Multiturn (25 bits)|Singleturn (13 bits)|Variable (set size in Frame Size)),edit,edit,edit
      mask CallbackString: ||el500x.modelChanged|||||EtherCATSlave.updateCustomDCEnable()|||||||||||||||||||||||||||||||
      mask TabNameString: Main,Main,Main,Main,Main,Main,Main,Distributed Clocks,Distributed Clocks,Distributed Clocks,Distributed Clocks,Distributed Clocks,Distributed Clocks,Distributed Clocks,Distributed Clocks,Distributed Clocks,Distributed Clocks,Distributed Clocks,CoE #x8000,CoE #x8000,CoE #x8000,CoE #x8000,CoE #x8000,CoE #x8000,CoE #x8000,CoE #x8000,CoE #x8000,CoE #x8000,CoE #x8000,CoE #x8010,CoE #x8010,CoE #x8010,CoE #x8010,CoE #x8010,CoE #x8010,CoE #x8010,CoE #x8010,CoE #x8010,CoE #x8010
      mask Display: disp('EL5001\nM:0 Idx:1')
  EL5021_0 : S-Function  LoadFcn=el5021().checkModelName()  FunctionName=ec_slave3  Parameters=Address,rv.SlaveConfig,rv.PortConfig,debug,tsample  SFunctionModules='ecrt_support'  EnableBusSupport=off  mask(EL5021){master=0, index=1, model=EL5021, revision=, tsample=-1, debug=0, dc_mode=FreeRun/SM-Synchron, dc_assign_activate=hex2dec('700'), dc_cycle0=0, dc_cycle0_factor=1, dc_shift0=-30600, dc_shift0_factor=0, dc_shift0_input=off, dc_cycle1=0, dc_cycle1_factor=1, dc_shift1=25000, dc_shift1_factor=0, sdo_01=off, sdo_02=off, sdo_03=on, sdo_04=on, sdo_05=10}
      mask prompts: index "Slave Index"; model "Device Model"; tsample "Sample Time (-1 inherited)"; dc_mode "Mode"; dc_assign_activate "Assign Activate"; dc_cycle0 "Cycle Time Sync 0"; dc_cycle0_factor "Factor"; dc_shift0 "Shift Time Sync0"; dc_shift0_factor "Factor"; dc_shift0_input "Shift Time0 Input"; dc_cycle1 "Cycle Time Sync1"; dc_cycle1_factor "Factor"; dc_shift1 "Shift Time Sync1"; dc_shift1_factor "Factor"; sdo_01 "8000:01 - Enable C reset"; sdo_02 "8000:0E - Reversion of rotation"; sdo_03 "8001:01 - Frequency error counter"; sdo_04 "8001:02 - Amplitude error counter"; sdo_05 "8001:11 - Analog resolution"
      mask help: Beckhoff EtherCAT 1Ch. Sin/Cos Encoder
      mask init:
      | Address = EtherCATSlave.formatAddress(master,index,tsample);
      | 
      | rv = el5021(model).configure(...
      |     [dc_mode, dc_assign_activate, ...
      |     dc_cycle0, dc_cycle0_factor,...
      |     dc_shift0, dc_shift0_factor, dc_shift0_input,...
      |     dc_cycle1, dc_cycle1_factor,...
      |     dc_shift1, dc_shift1_factor], ...
      |     [sdo_01, sdo_02, sdo_03, sdo_04, sdo_05]);
      |  
      | EtherCATSlave.setPortNames(...
      |     {rv.PortConfig.input.portname},...
      |     {rv.PortConfig.output.portname});
      | 
      | set_param(gcb,'AttributesFormatString',...
      |     sprintf('%s\nM:%i Idx:%s',...
      |             model,master,mat2str(index)))
      settings: AttributesFormatString=|
      | EL5021
      | M:0 Idx:1
      mask Help: web(etherlab_help_path('el5021.html'), '-helpbrowser');
      mask StyleString: edit,edit,popup(EL5021),edit,edit,edit,popup(FreeRun/SM-Synchron|DC-Synchron|DC-Synchron (input based)|Custom),edit,min,max,min,max,checkbox,min,max,min,max,checkbox,checkbox,checkbox,checkbox,edit
      mask CallbackString: ||el5021().updateRevision||||EtherCATSlave.updateCustomDCEnable();|||||||||||||||
      mask TabNameString: Main,Main,Main,Main,Main,Main,Distributed Clocks,Distributed Clocks,Distributed Clocks,Distributed Clocks,Distributed Clocks,Distributed Clocks,Distributed Clocks,Distributed Clocks,Distributed Clocks,Distributed Clocks,Distributed Clocks,CoE #x800x,CoE #x800x,CoE #x800x,CoE #x800x,CoE #x800x
      mask Display:
      | port_label('input', 1, 'bool[2]')
      | port_label('input', 2, 'Value')
      | port_label('output', 1, 'bool[5]')
      | port_label('output', 2, 'Counter')
      | port_label('output', 3, 'Latch')
  EL5101_0 : S-Function  LoadFcn=|  FunctionName=ec_slave3  Parameters=Address,rv.SlaveConfig,rv.PortConfig,debug,tsample  SFunctionModules='ecrt_support'  EnableBusSupport=off  mask(EL5101){master=0, index=1, model=EL5101, dcmode=FreeRun/SM-Synchron, x1601=off, x1602=off, x1603=on, x1A01=off, x1A02=off, x1A03=on, x1A04=off, x1A05=off, x1A06=off, x1A07=off, x1A08=off, tsample=0, debug=0, n8000_01=off, n8000_02=off, n8000_03=off, n8000_04=on, n8000_05=off, n8001_01=100, n8001_02=65535, x8010_01=off, x8010_02=off, x8010_03=off, x8010_04=Enable pos. gate, x8010_08=on, x8010_0A=off, x8010_0B=on, x8010_0C=on, x8010_0D=off, x8010_0E=off, x8010_10=on, x8010_11=10000, x8010_13=100, x8010_14=100, x8010_15=100, x8010_16=500, x8010_17=1600}
      | el5101('check')
      | if ~strcmp(bdroot(gcb),'etherlab_lib')
      |   disp([gcb ' is obsolete. Please replace'])
      | end
      mask prompts: index "Slave Index"; model "Device Model"; dcmode "DC Mode"; x1601 "RxPdo #x1601 (Excl 1602,1603)"; x1602 "RxPdo #x1602 (Excl 1601,1603)"; x1603 "RxPdo #x1603 (Excl 1601,1602)"; x1A01 "TxPdo #x1a01 (Excl 1a03,1a04,1a05,1a06,1a07,1a08)"; x1A02 "TxPdo #x1a02 (Excl 1a03,1a04,1a05,1a06,1a07,1a08)"; x1A03 "TxPdo #x1a03 (Excl 1a01,1a02,1a04)"; x1A04 "TxPdo #x1a04 (Excl 1a01,1a02,1a03)"; x1A05 "TxPdo #x1a05 (Excl 1a01,1a02,1a06)"; x1A06 "TxPdo #x1a06 (Excl 1a01,1a02,1a05)"; x1A07 "TxPdo #x1a07 (Excl 1a01,1a02,1a08)"; x1A08 "TxPdo #x1a08 (Excl 1a01,1a02,1a07)"; tsample "Sample Time (-1 inherited)"; n8000_01 "8000:01 - Enable Register Reload"; n8000_02 "8000:02 - Enable Index Reset"; n8000_03 "8000:03 - Enable FWD Count"; n8000_04 "8000:04 - Enable Positive Gate"; n8000_05 "8000:05 - Enable Negaitive Gate"; n8001_01 "8001:01 - Frequency Window"; n8001_02 "8001:02 - Counter Reload Value"; x8010_01 "8010:01 - Enable C reset"; x8010_02 "8010:02 - Enable extern reset"; x8010_03 "8010:03 - Enable up/down counter"; x8010_04 "8010:04 - Gate polarity"; x8010_08 "8010:08 - Disable filter"; x8010_0A "8010:0A - Enable micro increments"; x8010_0B "8010:0B - Open cct det A"; x8010_0C "8010:0C - Open cct det B"; x8010_0D "8010:0D - Open cct det C"; x8010_0E "8010:0E - Reversion of rotation"; x8010_10 "8010:10 - Extern Reset polarity"; x8010_11 "8010:11 - Frequency window"; x8010_13 "8010:13 - Frequency scaling"; x8010_14 "8010:14 - Period scaling"; x8010_15 "8010:15 - Frequency resolution"; x8010_16 "8010:16 - Period resolution"; x8010_17 "8010:17 - Frequency Wait Time"
      mask help: Beckhoff EtherCAT Incremental Encoder Input
      mask init:
      | Address = EtherCATSlave.formatAddress(master,index,tsample);
      | 
      | el5101('set');
      | rv = get_param(gcbh,'UserData');
      | rv.SlaveConfig.sdo = {...
      |     hex2dec('1011'), 1,32,hex2dec('64616f6c');
      |     hex2dec('8000'), 1, 8,n8000_01;
      |     hex2dec('8000'), 2, 8,n8000_02;
      |     hex2dec('8000'), 3, 8,n8000_03;
      |     hex2dec('8000'), 4, 8,n8000_04;
      |     hex2dec('8000'), 5, 8,n8000_05;
      |     hex2dec('8001'), 1,16,n8001_01;
      |     hex2dec('8001'), 2,16,n8001_02;
      |     hex2dec('8010'), 1, 8,x8010_01;
      |     hex2dec('8010'), 2, 8,x8010_02;
      |     hex2dec('8010'), 3, 8,x8010_03;
      |     hex2dec('8010'), 4, 8,x8010_04-1;
      |     hex2dec('8010'), 8, 8,x8010_08;
      |     hex2dec('8010'),10, 8,x8010_0A;
      |     hex2dec('8010'),11, 8,x8010_0B;
      |     hex2dec('8010'),12, 8,x8010_0C;
      |     hex2dec('8010'),13, 8,x8010_0D;
      |     hex2dec('8010'),14, 8,x8010_0E;
      |     hex2dec('8010'),16, 8,x8010_10;
      |     hex2dec('8010'),17,16,x8010_11;
      |     hex2dec('8010'),19,16,x8010_13;
      |     hex2dec('8010'),20,16,x8010_14;
      |     hex2dec('8010'),21,16,x8010_15;
      |     hex2dec('8010'),22,16,x8010_16;
      |     hex2dec('8010'),23,16,x8010_17;
      | };
      mask Help: web(etherlab_help_path('el5101.html'), '-helpbrowser');
      mask StyleString: edit,edit,popup(EL5101|EL5101-1006),popup(FreeRun/SM-Synchron|DC-Synchron|DC-Synchron (input based)),checkbox,checkbox,checkbox,checkbox,checkbox,checkbox,checkbox,checkbox,checkbox,checkbox,checkbox,edit,edit,checkbox,checkbox,checkbox,checkbox,checkbox,edit,edit,checkbox,checkbox,checkbox,popup(Disable gate|Enable pos. gate|Enable neg. gate),checkbox,checkbox,checkbox,checkbox,checkbox,checkbox,checkbox,edit,edit,edit,edit,edit,edit
      mask CallbackString: ||||el5101('ui')|el5101('ui')|el5101('ui')|el5101('ui')|el5101('ui')|el5101('ui')|el5101('ui')|el5101('ui')|el5101('ui')|el5101('ui')|el5101('ui')||||||||||||||||||||||||||
      mask TabNameString: Main,Main,Main,Main,Main,Main,Main,Main,Main,Main,Main,Main,Main,Main,Main,Main,Main,CoE #x8000,CoE #x8000,CoE #x8000,CoE #x8000,CoE #x8000,CoE #x8001,CoE #x8001,CoE #x8010,CoE #x8010,CoE #x8010,CoE #x8010,CoE #x8010,CoE #x8010,CoE #x8010,CoE #x8010,CoE #x8010,CoE #x8010,CoE #x8010,CoE #x8010,CoE #x8010,CoE #x8010,CoE #x8010,CoE #x8010,CoE #x8010
      mask Display: fprintf('%s\nIncr.-Enc\nM:%i Idx:%s', model, master, mat2str(index))
  EL5101_0010_0 : S-Function  LoadFcn=|  FunctionName=ec_slave3  Parameters=Address,rv.SlaveConfig,rv.PortConfig,debug,tsample  SFunctionModules='ecrt_support'  EnableBusSupport=off  mask(EL5101-0010){master=0, index=1, model=EL5101-0010, dcmode=FreeRun/SM-Synchron, x1600=on, x1601=off, x1A00=on, x1A01=off, x1A02=off, x1A03=off, x1A04=off, x1A05=off, tsample=0, debug=0, x8000_01=off, x8000_02=off, x8000_04=Enable pos. gate, x8000_0B=on, x8000_0C=on, x8000_0D=off, x8000_0E=off, x8000_10=on, x8000_11=10000, x8000_13=100, x8000_14=100, x8000_15=100, x8000_16=100, x8000_17=400}
      | el5101_0010('check')
      | if ~strcmp(bdroot(gcb),'etherlab_lib')
      |   disp([gcb ' is obsolete. Please replace'])
      | end
      mask prompts: index "Slave Index"; model "Device Model"; dcmode "DC Mode"; x1600 "RxPdo #x1600 (Excl 1601)"; x1601 "RxPdo #x1601 (Excl 1600)"; x1A00 "TxPdo #x1a00 (Excl 1a01)"; x1A01 "TxPdo #x1a01 (Excl 1a00)"; x1A02 "TxPdo #x1a02 (Excl 1a03)"; x1A03 "TxPdo #x1a03 (Excl 1a02)"; x1A04 "TxPdo #x1a04 (Excl 1a05)"; x1A05 "TxPdo #x1a05 (Excl 1a04)"; tsample "Sample Time (-1 inherited)"; x8000_01 "8000:01 - Enable C reset"; x8000_02 "8000:02 - Enable extern reset"; x8000_04 "8000:04 - Gate polarity"; x8000_0B "8000:0B - Open cct det A"; x8000_0C "8000:0C - Open cct det B"; x8000_0D "8000:0D - Open cct det C"; x8000_0E "8000:0E - Reversion of rotation"; x8000_10 "8000:10 - Extern Reset polarity"; x8000_11 "8000:11 - Frequency window"; x8000_13 "8000:13 - Frequency scaling"; x8000_14 "8000:14 - Period scaling"; x8000_15 "8000:15 - Frequency resolution"; x8000_16 "8000:16 - Period resolution"; x8000_17 "8000:17 - Frequency Wait Time"
      mask help: Beckhoff EtherCAT Incremental Encoder Input
      mask init:
      | Address = EtherCATSlave.formatAddress(master,index,tsample);
      | 
      | el5101_0010('set');
      | rv = get_param(gcbh,'UserData');
      | rv.SlaveConfig.sdo = {...
      |     hex2dec('1011'), 1,32,hex2dec('64616f6c');
      |     hex2dec('8000'), 1, 8,x8000_01;
      |     hex2dec('8000'), 2, 8,x8000_02;
      |     hex2dec('8000'), 4, 8,x8000_04-1;
      |     hex2dec('8000'),11, 8,x8000_0B;
      |     hex2dec('8000'),12, 8,x8000_0C;
      |     hex2dec('8000'),13, 8,x8000_0D;
      |     hex2dec('8000'),14, 8,x8000_0E;
      |     hex2dec('8000'),16, 8,x8000_10;
      |     hex2dec('8000'),17,16,x8000_11;
      |     hex2dec('8000'),19,16,x8000_13;
      |     hex2dec('8000'),20,16,x8000_14;
      |     hex2dec('8000'),21,16,x8000_15;
      |     hex2dec('8000'),22,16,x8000_16;
      |     hex2dec('8000'),23,16,x8000_17;
      | };
      mask Help: web(etherlab_help_path('el5101-0010.html'), '-helpbrowser');
      mask StyleString: edit,edit,popup(EL5101-0010),popup(FreeRun/SM-Synchron|DC-Synchron|DC-Synchron (input based)),checkbox,checkbox,checkbox,checkbox,checkbox,checkbox,checkbox,checkbox,edit,edit,checkbox,checkbox,popup(Disable gate|Enable pos. gate|Enable neg. gate),checkbox,checkbox,checkbox,checkbox,checkbox,edit,edit,edit,edit,edit,edit
      mask CallbackString: ||||el5101_0010('ui')|el5101_0010('ui')|el5101_0010('ui')|el5101_0010('ui')|el5101_0010('ui')|el5101_0010('ui')|el5101_0010('ui')|el5101_0010('ui')||||||||||||||||
      mask TabNameString: Main,Main,Main,Main,Main,Main,Main,Main,Main,Main,Main,Main,Main,Main,CoE #x8000,CoE #x8000,CoE #x8000,CoE #x8000,CoE #x8000,CoE #x8000,CoE #x8000,CoE #x8000,CoE #x8000,CoE #x8000,CoE #x8000,CoE #x8000,CoE #x8000,CoE #x8000
      mask Display: fprintf('%s\nIncr.-Enc\nM:%i Idx:%s', model, master, mat2str(index))
  EL515x_1 : S-Function  LoadFcn=|  FunctionName=ec_slave3  Parameters=Address,rv.SlaveConfig,rv.PortConfig,debug,tsample  SFunctionModules='ecrt_support'  EnableBusSupport=off  mask(EL515x){master=0, index=1, model=EL5152, dcmode=FreeRun/SM-Synchron, x1600=on, x1601=off, x1602=off, x1603=off, x1A00=on, x1A01=off, x1A02=off, x1A03=off, x1A04=off, x1A05=off, x1A06=off, x1A07=off, tsample=0, debug=0, x8000_01=off, x8000_02=off, x8000_03=off, x8000_04=Enable pos. gate, x8000_08=off, x8000_0A=off, x8000_0E=off, x8000_0F=off, x8000_10=on, x8000_11=10000, x8000_13=100, x8000_14=100, x8000_15=100, x8000_16=100, x8000_17=1600, x8010_03=off, x8010_08=off, x8010_0A=off, x8010_0E=off, x8010_0F=off, x8010_11=10000, x8010_13=100, x8010_14=100, x8010_15=100, x8010_16=100, x8010_17=1600}
      | el515x('check')
      | if ~strcmp(bdroot(gcb),'etherlab_lib')
      |   disp([gcb ' is obsolete. Please replace'])
      | end
      mask prompts: index "Slave Index"; model "Device Model"; dcmode "DC Mode"; x1600 "RxPdo #x1600 (Excl 1601)"; x1601 "RxPdo #x1601 (Excl 1600)"; x1602 "RxPdo #x1602 (Excl 1603)"; x1603 "RxPdo #x1603 (Excl 1602)"; x1A00 "TxPdo #x1a00 (Excl 1a01)"; x1A01 "TxPdo #x1a01 (Excl 1a00)"; x1A02 "TxPdo #x1a02 (Excl 1a03)"; x1A03 "TxPdo #x1a03 (Excl 1a02)"; x1A04 "TxPdo #x1a04 (Excl 1a05)"; x1A05 "TxPdo #x1a05 (Excl 1a04)"; x1A06 "TxPdo #x1a06 (Excl 1a07)"; x1A07 "TxPdo #x1a07 (Excl 1a06)"; tsample "Sample Time (-1 inherited)"; x8000_01 "8000:01 - Enable C reset"; x8000_02 "8000:02 - Enable extern reset"; x8000_03 "8000:03 - Enable up/down counter"; x8000_04 "8000:04 - Gate polarity"; x8000_08 "8000:08 - Disable filter"; x8000_0A "8000:0A - Enable micro increments"; x8000_0E "8000:0E - Reversion of rotation"; x8000_0F "8000:0F - Freqency window in ms"; x8000_10 "8000:10 - Extern Reset polarity"; x8000_11 "8000:11 - Frequency window"; x8000_13 "8000:13 - Frequency scaling"; x8000_14 "8000:14 - Period scaling"; x8000_15 "8000:15 - Frequency resolution"; x8000_16 "8000:16 - Period resolution"; x8000_17 "8000:17 - Frequency Wait Time"; x8010_03 "8010:03 - Enable up/down counter"; x8010_08 "8010:08 - Disable filter"; x8010_0A "8010:0A - Enable micro increments"; x8010_0E "8010:0E - Reversion of rotation"; x8010_0F "8010:0F - Freqency window in ms"; x8010_11 "8010:11 - Frequency window"; x8010_13 "8010:13 - Frequency scaling"; x8010_14 "8010:14 - Period scaling"; x8010_15 "8010:15 - Frequency resolution"; x8010_16 "8010:16 - Period resolution"; x8010_17 "8010:17 - Frequency Wait Time"
      mask help: Beckhoff EtherCAT Incremental Encoder Input
      mask init:
      | Address = EtherCATSlave.formatAddress(master,index,tsample);
      | 
      | el515x('set');
      | rv = get_param(gcbh,'UserData');
      | rv.SlaveConfig.sdo = {...
      |     hex2dec('8000'), 3, 8,x8000_03;
      |     hex2dec('8000'), 8, 8,x8000_08;
      |     hex2dec('8000'),10, 8,x8000_0A;
      |     hex2dec('8000'),14, 8,x8000_0E;
      |     hex2dec('8000'),15, 8,x8000_0F;
      |     hex2dec('8000'),17,16,x8000_11;
      |     hex2dec('8000'),19,16,x8000_13;
      |     hex2dec('8000'),20,16,x8000_14;
      |     hex2dec('8000'),21,16,x8000_15;
      |     hex2dec('8000'),22,16,x8000_16;
      |     hex2dec('8000'),23,16,x8000_17;
      | };
      | 
      | if strncmp(model,'EL5151',6)
      |     rv.SlaveConfig.sdo = vertcat(rv.SlaveConfig.sdo,...
      |         { hex2dec('8000'), 1, 8,x8000_01;
      |           hex2dec('8000'), 2, 8,x8000_02;
      |           hex2dec('8000'), 4, 8,x8000_04;
      |           hex2dec('8000'),16, 8,x8000_10});
      | else
      |     rv.SlaveConfig.sdo = vertcat(rv.SlaveConfig.sdo,...
      |         { hex2dec('8010'), 3, 8,x8010_03;
      |           hex2dec('8010'), 8, 8,x8010_08;
      |           hex2dec('8010'),10, 8,x8010_0A;
      |           hex2dec('8010'),14, 8,x8010_0E;
      |           hex2dec('8010'),15, 8,x8010_0F;
      |           hex2dec('8010'),17,16,x8010_11;
      |           hex2dec('8010'),19,16,x8010_13;
      |           hex2dec('8010'),20,16,x8010_14;
      |           hex2dec('8010'),21,16,x8010_15;
      |           hex2dec('8010'),22,16,x8010_16;
      |           hex2dec('8010'),23,16,x8010_17});
      | end
      mask Help: web(etherlab_help_path('el515x.html'), '-helpbrowser');
      mask StyleString: edit,edit,popup(EL5151|EL5151-0080|EL5152),popup(FreeRun/SM-Synchron|DC-Synchron|DC-Synchron (input based)),checkbox,checkbox,checkbox,checkbox,checkbox,checkbox,checkbox,checkbox,checkbox,checkbox,checkbox,checkbox,edit,edit,checkbox,checkbox,checkbox,popup(Disable gate|Enable pos. gate|Enable neg. gate),checkbox,checkbox,checkbox,checkbox,checkbox,edit,edit,edit,edit,edit,edit,checkbox,checkbox,checkbox,checkbox,checkbox,edit,edit,edit,edit,edit,edit
      mask CallbackString: ||el515x('ui')||el515x('ui')|el515x('ui')|el515x('ui')|el515x('ui')|el515x('ui')|el515x('ui')|el515x('ui')|el515x('ui')|el515x('ui')|el515x('ui')|el515x('ui')|el515x('ui')||||||||||||||||||||||||||||
      mask TabNameString: Main,Main,Main,Main,Main,Main,Main,Main,Main,Main,Main,Main,Main,Main,Main,Main,Main,Main,CoE #x8000,CoE #x8000,CoE #x8000,CoE #x8000,CoE #x8000,CoE #x8000,CoE #x8000,CoE #x8000,CoE #x8000,CoE #x8000,CoE #x8000,CoE #x8000,CoE #x8000,CoE #x8000,CoE #x8000,CoE #x8010,CoE #x8010,CoE #x8010,CoE #x8010,CoE #x8010,CoE #x8010,CoE #x8010,CoE #x8010,CoE #x8010,CoE #x8010,CoE #x8010
      mask Display: fprintf('%s\nIncr.-Enc\nM:%i Idx:%s', model, master, mat2str(index))
  EL51xx_0 : S-Function  LoadFcn=el51xx().checkModelName()  FunctionName=ec_slave3  Parameters=Address,rv.SlaveConfig,rv.PortConfig,debug,tsample  SFunctionModules='ecrt_support'  EnableBusSupport=off  mask(EL51xx){master=0, index=1, model=EL5101, revision=, pdo_x1600=off, pdo_x1601=on, pdo_x1602=off, pdo_x1603=off, pdo_x1A00=off, pdo_x1A01=on, pdo_x1A02=off, pdo_x1A03=off, pdo_x1A04=off, pdo_x1A05=off, pdo_x1A06=off, pdo_x1A07=off, tsample=-1, debug=0, dc_mode=FreeRun/SM-Synchron, dc_assign_activate=hex2dec('320')    % EL51x1: '320'; El5152: '720', dc_cycle0=0, dc_cycle0_factor=1, dc_shift0=0, dc_shift0_factor=0, dc_shift0_input=off, dc_cycle1=0, dc_cycle1_factor=1, dc_shift1=0, dc_shift1_factor=0, sdo_01=off, sdo_02=off, sdo_03=off, sdo_04=on, sdo_05=off, sdo_06=off, sdo_07=off, sdo_08=off, sdo_09=Enable pos. gate, sdo_10=off, sdo_11=off, sdo_12=on, sdo_13=on, sdo_14=off, sdo_15=off, sdo_16=us, sdo_17=Rising edge, sdo_18=10000, sdo_19=100, sdo_20=100, sdo_21=100, sdo_22=100, sdo_23=1600, sdo_24=100, sdo_25=65535, sdo_26=off, sdo_27=off, sdo_28=off, sdo_29=Enable pos. gate, sdo_30=off, sdo_31=off, sdo_32=on, sdo_33=on, sdo_34=off, sdo_35=off, sdo_36=us, sdo_37=Rising edge, sdo_38=10000, sdo_39=100, sdo_40=100, sdo_41=100, sdo_42=500, sdo_43=1600}
      mask prompts: index "Slave Index"; model "Device Model"; pdo_x1600 "RxPdo #x1600"; pdo_x1601 "RxPdo #x1601"; pdo_x1602 "RxPdo #x1602"; pdo_x1603 "RxPdo #x1603"; pdo_x1A00 "TxPdo #x1a00"; pdo_x1A01 "TxPdo #x1a01"; pdo_x1A02 "TxPdo #x1a02"; pdo_x1A03 "TxPdo #x1a03"; pdo_x1A04 "TxPdo #x1a04"; pdo_x1A05 "TxPdo #x1a05"; pdo_x1A06 "TxPdo #x1a06"; pdo_x1A07 "TxPdo #x1a07"; tsample "Sample Time (-1 inherited)"; dc_mode "DC Mode"; dc_assign_activate "Assign Activate"; dc_cycle0 "Cycle Time Sync 0 [ns]"; dc_cycle0_factor "Factor"; dc_shift0 "Shift Time Sync0 [ns]"; dc_shift0_factor "Factor"; dc_shift0_input "Shift Time0 Input"; dc_cycle1 "Cycle Time Sync1 [ns]"; dc_cycle1_factor "Factor"; dc_shift1 "Shift Time Sync1 [ns]"; dc_shift1_factor "Factor"; sdo_01 "8000:01 - Enable register reload"; sdo_02 "8000:02 - Enable index reset"; sdo_03 "8000:03 - Enable FWD count"; sdo_04 "8000:04 - Enable pos. gate"; sdo_05 "8000:05 - Enable neg. gate"; sdo_06 "8000:01 - Enable C reset"; sdo_07 "8000:02 - Enable extern reset"; sdo_08 "8000:03 - Enable up/down counter"; sdo_09 "8000:04 - Gate polarity"; sdo_10 "8000:08 - Disable filter"; sdo_11 "8000:0A - Enable micro increments"; sdo_12 "8000:0B - Open circuit detection A"; sdo_13 "8000:0C - Open circuit detection B"; sdo_14 "8000:0D - Open circuit detection C"; sdo_15 "8000:0E - Reversion of rotation"; sdo_16 "8000:0F - Frequency window base (8000:11)"; sdo_17 "8000:10 - Extern reset polarity"; sdo_18 "8000:11 - Frequency window"; sdo_19 "8000:13 - Frequency scaling [1/Hz]"; sdo_20 "8000:14 - Period scaling [ns]"; sdo_21 "8000:15 - Frequency resolution [1/Hz]"; sdo_22 "8000:16 - Period resolution [ns]"; sdo_23 "8000:17 - Frequency wait time [ms]"; sdo_24 "8001:01 - Frequency window [16us]"; sdo_25 "8001:02 - Counter reload value"; sdo_26 "8010:01 - Enable C reset"; sdo_27 "8010:02 - Enable extern reset"; sdo_28 "8010:03 - Enable up/down counter"; sdo_29 "8010:04 - Gate polarity"; sdo_30 "8010:08 - Disable filter"; sdo_31 "8010:0A - Enable micro increments"; sdo_32 "8010:0B - Open circuit detection A"; sdo_33 "8010:0C - Open circuit detection B"; sdo_34 "8010:0D - Open circuit detection C"; sdo_35 "8010:0E - Reversion of rotation"; sdo_36 "8010:0F - Frequency window base (8010:11)"; sdo_37 "8010:10 - Extern reset polarity"; sdo_38 "8010:11 - Frequency window"; sdo_39 "8010:13 - Frequency scaling [1/Hz]"; sdo_40 "8010:14 - Period scaling [ns]"; sdo_41 "8010:15 - Frequency resolution [1/Hz]"; sdo_42 "8010:16 - Period resolution [ns]"; sdo_43 "8010:17 - Frequency wait time [ms]"
      mask help: Beckhoff EtherCAT Incremental Encoder Input
      mask init:
      | Address = EtherCATSlave.formatAddress(master,index,tsample);
      | 
      | pdo = hex2dec({'1600', '1601', '1602', '1603',...
      |      '1A00', '1A01', '1A02', '1A03', '1A04', ...
      |      '1A05', '1A06', '1A07'});
      |      
      | rv = el51xx(model).configure(...
      |     pdo(boolean([pdo_x1600, pdo_x1601, pdo_x1602, ...
      |                  pdo_x1603, pdo_x1A00, pdo_x1A01, ...
      |                  pdo_x1A02, pdo_x1A03, pdo_x1A04, ...
      |                  pdo_x1A05, pdo_x1A06, pdo_x1A07])), ...
      |     [  sdo_01,   sdo_02,   sdo_03, sdo_04, sdo_05, sdo_06, sdo_07,... 
      |        sdo_08, sdo_09-1,   sdo_10, sdo_11, sdo_12, sdo_13, sdo_14,...
      |        sdo_15, sdo_16-1, sdo_17-1, sdo_18, sdo_19, sdo_20, sdo_21,...
      |        sdo_22,   sdo_23,   sdo_24, sdo_25, sdo_26, sdo_27, sdo_28,...
      |      sdo_29-1,   sdo_30,   sdo_31, sdo_32, sdo_33, sdo_34, sdo_35,...
      |      sdo_36-1, sdo_37-1,   sdo_38, sdo_39, sdo_40, sdo_41, sdo_42,...
      |        sdo_43],...
      |     [dc_mode, dc_assign_activate, ...
      |      dc_cycle0, dc_cycle0_factor,...
      |      dc_shift0, dc_shift0_factor, dc_shift0_input,...
      |      dc_cycle1, dc_cycle1_factor,...
      |      dc_shift1, dc_shift1_factor]);     
      | 
      | EtherCATSlave.setPortNames(...
      |     {rv.PortConfig.input.portname},...
      |     {rv.PortConfig.output.portname});
      | 
      | set_param(gcb,'AttributesFormatString',...
      |     sprintf('%s\nM:%i Idx:%s',...
      |             model,master,mat2str(index)))
      settings: AttributesFormatString=|
      | EL5101
      | M:0 Idx:1
      mask Help: web(etherlab_help_path('el51xx.html'), '-helpbrowser');
      mask StyleString: edit,edit,popup(EL5101|EL5101-0010|EL5151|EL5152|EL5152-0000-0016),edit,checkbox,checkbox,checkbox,checkbox,checkbox,checkbox,checkbox,checkbox,checkbox,checkbox,checkbox,checkbox,edit,edit,popup(FreeRun/SM-Synchron|DC-Synchron|DC-Synchron (input based)|Custom),edit,min,max,min,max,checkbox,min,max,min,max,checkbox,checkbox,checkbox,checkbox,checkbox,checkbox,checkbox,checkbox,popup(Disable gate|Enable pos. gate|Enable neg. gate),checkbox,checkbox,checkbox,checkbox,checkbox,checkbox,popup(us|ms),popup(Falling edge|Rising edge),edit,edit,edit,edit,edit,edit,edit,edit,checkbox,checkbox,checkbox,popup(Disable gate|Enable pos. gate|Enable neg. gate),checkbox,checkbox,checkbox,checkbox,checkbox,checkbox,popup(us|ms),popup(Falling edge|Rising edge),edit,edit,edit,edit,edit,edit
      mask CallbackString: ||el51xx.modelChanged||el51xx.updatePDO|el51xx.updatePDO|el51xx.updatePDO|el51xx.updatePDO|el51xx.updatePDO|el51xx.updatePDO|el51xx.updatePDO|el51xx.updatePDO|el51xx.updatePDO|el51xx.updatePDO|el51xx.updatePDO|el51xx.updatePDO|||EtherCATSlave.updateCustomDCEnable()|||||||||||||||||||||||||||||||||||||||||||||||||||||
      mask TabNameString: Main,Main,Main,Main,Main,Main,Main,Main,Main,Main,Main,Main,Main,Main,Main,Main,Main,Main,Distributed Clocks,Distributed Clocks,Distributed Clocks,Distributed Clocks,Distributed Clocks,Distributed Clocks,Distributed Clocks,Distributed Clocks,Distributed Clocks,Distributed Clocks,Distributed Clocks,CoE #x800x,CoE #x800x,CoE #x800x,CoE #x800x,CoE #x800x,CoE #x800x,CoE #x800x,CoE #x800x,CoE #x800x,CoE #x800x,CoE #x800x,CoE #x800x,CoE #x800x,CoE #x800x,CoE #x800x,CoE #x800x,CoE #x800x,CoE #x800x,CoE #x800x,CoE #x800x,CoE #x800x,CoE #x800x,CoE #x800x,CoE #x800x,CoE #x800x,CoE #x8010,CoE #x8010,CoE #x8010,CoE #x8010,CoE #x8010,CoE #x8010,CoE #x8010,CoE #x8010,CoE #x8010,CoE #x8010,CoE #x8010,CoE #x8010,CoE #x8010,CoE #x8010,CoE #x8010,CoE #x8010,CoE #x8010,CoE #x8010
      mask Display:
      | port_label('input', 1, 'Ctrl')
      | port_label('input', 2, 'Value')
      | port_label('output', 1, 'Status')
      | port_label('output', 2, 'Counter')
      | port_label('output', 3, 'Latch')
  EL9xxx_0 : S-Function  LoadFcn=el9xxx().checkModelName()  FunctionName=ec_slave3  Parameters=Address,rv.SlaveConfig,rv.PortConfig,debug,tsample  SFunctionModules='ecrt_support'  EnableBusSupport=off  mask(EL9xxx){master=0, index=1, model=EL9110, revision=, vector=off, tsample=0, debug=0}
      mask prompts: index "Slave Index"; model "Device Model"; vector "Vector Outputs"; tsample "Sample Time"; debug "Debug Level"
      mask help:
      | Beckhoff EtherCAT System Terminals
      | with diagnosis
      mask init:
      | Address = EtherCATSlave.formatAddress(master,index,tsample);
      | 
      | rv = el9xxx(model).configure(vector);
      mask Help: web(etherlab_help_path('el9xxx.html'), '-helpbrowser');
      mask StyleString: edit,edit,popup(EL9110|EL9160|EL9210|EL9210-0020|EL9260|EL9410|EL9505|EL9508|EL9510|EL9512|EL9515|EL9560),edit,checkbox,edit,edit
      mask CallbackString: ||el9xxx().updateRevision()||||
      mask Display: fprintf('%s\nM:%i Idx:%s', model, master, mat2str(index))
  EP1xxx_0 : S-Function  LoadFcn=ep1xxx().checkModelName()  FunctionName=ec_slave3  Parameters=Address,rv.SlaveConfig,rv.PortConfig,debug,tsample  SFunctionModules='ecrt_support'  EnableBusSupport=off  mask(EP1xxx){master=0, index=1, model=EP1008-0002, revision=, vector=on, tsample=0, debug=0}
      mask prompts: index "Slave Index"; model "Device Model"; vector "Vector Output"; tsample "Sample Time"; debug "Deug Level"
      mask help: Beckhoff EtherCAT Digital Input Fieldbus Box
      mask init:
      | Address = EtherCATSlave.formatAddress(master,index,tsample);
      | 
      | rv = ep1xxx(model).configure(vector);
      mask Help:
      | This block implements the Beckhoff's EtherCAT series of Digital Input Terminals.
      | <p/>
      | Choose or set the following options:
      | <h4>Master:</h4>
      | Set the EtherCAT Master number that this terminal is connected to.
      | 
      | <h4>Slave Index:</h4>
      | Set the EtherCAT slave index. Following address formats are allowed:
      | <ol>
      | <li> Absolute addressing: a scalar number <<b><tt>n</tt></b>> representing the (zero based) absolute position in the bus.
      | <li> SSId addressing: the Secondary Slave (or 'Alias') Addressing has the form <<b><tt>[alias position]</tt></b>> where <b><tt>alias</tt></b> is the Secondary Slave Id of the EtherCAT slave and <b><tt>position</tt></b> is the offset after the slave with the given <b><tt>alias</tt></b>. The SSId has to be preprogrammed into the slave with other service tools (see 'ethercat alias --help').
      | </ol>
      | 
      | <h4> Device Model</h4>
      | Select the model that is used. This sets the number of outputs of this block.
      | 
      | <h4>Output Type</h4>
      | The block output type corresponding to the terminal inputs can be one of the following:
      | <ul>
      | <li><b>Vector Output</b>: This sets one output vector with a width equal to the number of digital inputs to the terminal.
      | <li><b>Separate Outputs</b>: This sets the number of outputs corresponding to the digital inputs to the terminal.
      | </ul>
      | 
      | <h4>Sample Time</h4>
      | Select the correct sample time. Setting this to 0 makes for a sample time at the model's base rate. If another block can set the sample time, choose -1 for inherited sample time.
      mask StyleString: edit,edit,popup(EP1008-0001|EP1008-0002|EP1008-0022|EP1018-0001|EP1018-0002|EP1098-0001|EP1111|EP1122-0001|EP1809-0021|EP1809-0022|EP1819-0021|EP1819-0022),edit,checkbox,edit,edit
      mask CallbackString: ||ep1xxx().updateRevision()||||
      mask Display: fprintf('%s\nM:%i Idx:%s', model, master, mat2str(index))
  EP2xxx_0 : S-Function  LoadFcn=ep2xxx().checkModelName()  FunctionName=ec_slave3  Parameters=Address,rv.SlaveConfig,rv.PortConfig,debug,tsample  SFunctionModules='ecrt_support'  EnableBusSupport=off  mask(EP2xxx){master=0, index=1, model=EP2001-1000, revision=, vector=on, tsample=-1, debug=0}
      mask prompts: index "Slave Index"; model "Device Model"; vector "Vector Input"; tsample "Sample Time"; debug "Debug Level"
      mask help: Beckhoff EtherCAT Digital Output Fieldbus Box
      mask init:
      | Address = EtherCATSlave.formatAddress(master,index,tsample);
      | 
      | rv = ep2xxx(model).configure(vector);
      mask Help:
      | This block implements the Beckhoff's EtherCAT series of Digital Input Terminals.
      | <p/>
      | Choose or set the following options:
      | <h4>Master:</h4>
      | Set the EtherCAT Master number that this terminal is connected to.
      | 
      | <h4>Slave Index:</h4>
      | Set the EtherCAT slave index. Following address formats are allowed:
      | <ol>
      | <li> Absolute addressing: a scalar number <<b><tt>n</tt></b>> representing the (zero based) absolute position in the bus.
      | <li> SSId addressing: the Secondary Slave (or 'Alias') Addressing has the form <<b><tt>[alias position]</tt></b>> where <b><tt>alias</tt></b> is the Secondary Slave Id of the EtherCAT slave and <b><tt>position</tt></b> is the offset after the slave with the given <b><tt>alias</tt></b>. The SSId has to be preprogrammed into the slave with other service tools (see 'ethercat alias --help').
      | </ol>
      | 
      | <h4> Device Model</h4>
      | Select the model that is used. This sets the number of outputs of this block.
      | 
      | <h4>Output Type</h4>
      | The block output type corresponding to the terminal inputs can be one of the following:
      | <ul>
      | <li><b>Vector Output</b>: This sets one output vector with a width equal to the number of digital inputs to the terminal.
      | <li><b>Separate Outputs</b>: This sets the number of outputs corresponding to the digital inputs to the terminal.
      | </ul>
      | 
      | <h4>Sample Time</h4>
      | Select the correct sample time. Setting this to 0 makes for a sample time at the model's base rate. If another block can set the sample time, choose -1 for inherited sample time.
      mask StyleString: edit,edit,popup(EP2001-1000|EP2008-0001|EP2008-0002|EP2008-0022|EP2028-0001|EP2028-0002|EP2028-0032|EP2308-0000|EP2308-0001|EP2308-0002|EP2316-0003|EP2316-0008|EP2318-0001|EP2318-0002|EP2328-0001|EP2328-0002|EP2338-0001|EP2338-0002|EP2338-1001|EP2338-1002|EP2339-0021|EP2339-0022|EP2349-0021|EP2349-0022|EP2624|EP2624-0002|EP2809-0021|EP2809-0022),edit,checkbox,edit,edit
      mask CallbackString: ||ep2xxx().updateRevision()||||
      mask Display: fprintf('%s\nM:%i Idx:%s', model, master, mat2str(index))
  EP31xx_0 : S-Function  LoadFcn=|  FunctionName=ec_slave3  Parameters=Address,rv.SlaveConfig,rv.PortConfig,debug,tsample  SFunctionModules='ecrt_support'  EnableBusSupport=off  mask(EP3xxx){master=0, index=1, model=EP3174-0002, type_1=-10...+10 V, type_2=-10...+10 V, type_3=-10...+10 V, type_4=-10...+10 V, dc=FreeRun/SM-Synchron, dccustomer=[1 hex2dec('700') 0 0 0 0 0 0 0], vector=on, raw=off, scale=1, offset=0, tau=1, status=off, tsample=0, debug=0}
      | ep31xx('check')
      | if ~strcmp(bdroot(gcb),'etherlab_lib')
      |   disp([gcb ' is obsolete. Please replace'])
      | end
      mask prompts: index "Slave Index"; model "Device Model"; type_1 "Channel 1 Type"; type_2 "Channel 2 Type"; type_3 "Channel 3 Type"; type_4 "Channel 4 Type"; dc "DC Mode"; dccustomer "Dc Customer"; vector "Vector Ports"; raw "Raw Bits"; scale "Output Scale (empty for none)"; offset "Output Offset (empty for none)"; tau "LPF Time Constant (sec)"; status "Status Output"; tsample "Sample Time (-1 for inherited)"
      mask help: Beckhoff Analog Input 16-Bit Fieldbus Box
      mask init:
      | Address = EtherCATSlave.formatAddress(master,index,tsample);
      | 
      | ep31xx('set');  % Report errors
      | 
      | rv = get_param(gcbh,'UserData');
      mask Help:
      | This block generically implements the EtherCAT 16-Bit Analog Input Fieldbus box Terminal for various models.
      | <p/>
      | The block input is generally a <tt>double</tt> from the range 0..1 for unipolar terminals and -1..1 for bipolar terminals, where 1 is the highest possible output of the terminal.
      | <p/>
      | Exceeding the input range simply saturates the terminal's output.
      | <p/>
      | The following Terminals are supported:
      | <center>
      | <table width="80%">
      | <tr><td>EP3174</td><td>4 port differential input</td></tr>
      | <tr><td>EP3182</td><td>2 port single ended input</td></tr>
      | <tr><td>EP3184</td><td>4 port single ended input</td></tr>
      | </table>
      | </center>
      | <p/>
      | Choose and set the following options:
      | <h4>Master:</h4>
      | Set the EtherCAT Master of this terminal.
      | 
      | <h4>Slave Index:</h4>
      | Set the EtherCAT slave index. Following address formats are allowed:
      | <ol>
      | <li> Absolute addressing: a scalar number <<b><tt>n</tt></b>> representing the (zero based) absolute position in the bus.
      | <li> SSId addressing: the Secondary Slave (or 'Alias') Addressing has the form <<b><tt>[alias position]</tt></b>> where <b><tt>alias</tt></b> is the Secondary Slave Id of the EtherCAT slave and <b><tt>position</tt></b> is the offset after the slave with the given <b><tt>alias</tt></b>. The SSId has to be preprogrammed into the slave with other service tools (see 'ethercat alias --help').
      | </ol>
      | 
      | <h4>Device Model:</h4>
      | Choose the device at the Indexed position of the master.
      | 
      | <h4>Channel 1-4 Type:</h4>
      | Choose the output type of the channel.
      | 
      | <h4>DC Mode:</h4>
      | Choose the DC Mode for the module.
      | 
      | <h4>DC Customer:</h4>
      | Do customized DC Settings in a vector
      | <<b><tt>[AssignActivate, CycleTimeSync0, CycleTimeSync0Factor, ShiftTimeSync0, ShiftTimeSync0Factor, ...
      | ShiftTimeSync0Input, CycleTimeSync1, CycleTimeSync1Factor, ShiftTimeSync1, ShiftTimeSync1Factor]</tt></b>>
      | 
      | <ul>
      | <li><<b><tt>AssignActivate:</tt></b>> Value for DC-mode setting
      | <li><<b><tt>CycleTimeSync0:</tt></b>> CycleTimeSync0 Value
      | <li><<b><tt>CycleTimeSync0Factor:</tt></b>> 1 or 0. If CycleTimeSync0Factor equals one the cycletimesync0 value is internally set to the process cycletime.
      | <li><<b><tt>ShiftTimeSync0:</tt></b>> ShiftTimeSync0 Value
      | <li><<b><tt>ShiftTimeSync0Factor:</tt></b>> 1 or 0. If ShiftTimeSync0Factor equals one the Slave is synced on the input event
      | <li><<b><tt>ShiftTimeSync0Input:</tt></b>> 1 or 0. If ShiftTimeSync0Input equals one the Slave is synced on the input event
      | <li><<b><tt>CycleTimeSync1:</tt></b>> CycleTimeSync1 Value
      | <li><<b><tt>CycleTimeSync1Factor:</tt></b>> 1 or 0. If CycleTimeSync1Factor equals one the CycletTimesSync1 value is internally set to the process cycletime.
      | <li><<b><tt>ShiftTimeSync1:</tt></b>>ShiftTimeSync1 Value
      | <li><<b><tt>ShiftTimeSync1Factor:</tt></b>> ShiftTimeSync1Factor Value
      | </ul>
      | 
      | <h4>Output Type:</h4>
      | <ul>
      | <li>Choose <b>Vector Output</b> to have a single output as a vector
      | with a size corresponding to the channel count of the terminal. This mode also allows a status output port to be displayed. <br/>
      | <li>Choose <b>Separate Outputs</b> to have one output for every channel.
      | </ul>
      | <h4>Output Full Scale</h4>
      | When <b>Output Data Type</b> is set to <b>Double with scale and offset</b>, the block's output value at full scale terminal input can be set here.
      | 
      | <h4>Output Offset</h4>
      | When <b>Output Data Type</b> is set to <b>Double with scale and offset</b>, the blocks output at zero terminal input can be set here. Note that the Full Scale above is also increased by this amount. Note furthermore that this corresponds to the minimum input for terminals such as 4..20mA.
      | 
      | <h4>Output Data Type</h4>
      | Choose the block's output data type for the output signal. Available are:
      | <ul>
      | <li><b><tt>Raw</tt></b> outputting the internal raw value as <tt>int16_T</tt> or <tt>uint16_T</tt> as appropriate
      | <li><b><tt>Double</tt></b> outputting 0..10, -10..10, 0..0.02 and 0.004..0.02 depending on the Model as appropriate
      | <li><b><tt>Double with scale and offset</tt></b>, allowing the output to be scaled with an offset.
      | </ul>
      | 
      | <p>
      | Choosing <b>Status Output</b> provides a port of type <tt>uint8_T</tt> where the status is presented. This is only enabled when <b>Vector Output</b> is selected. Terminal input over- and underrange can be detected using this output. See the terminal's documentation.
      | 
      | <h4>Output Filter</h4>
      | When not in <b>Raw</b> mode, the <b>Output Filter</b> checkbox becomes available, allowing the use of an internal low pass filter. Enter the <b>LPF Time Constant</b> for the filter in the field below.
      | <br>For continuous sample time systems (0 in Sample Time), the filter is also continuous. Discrete samples systems (Sample Time > 0) uses an equivalent discrete low pass filter with a similar time constant.
      | 
      | <p>
      | Set the <b>Sample Time</b> for the block. <tt>0</tt> is continuous sample time (runs at the model's base rate). Setting <tt>-1</tt> will try to set the time using back propagation.
      mask StyleString: edit,edit,popup(EP3174-0002|EP3182-1002|EP3184-0002|EP3184-1002),popup(-10...+10 V|0...20 mA|4...20 mA|0...10 V),popup(-10...+10 V|0...20 mA|4...20 mA|0...10 V),popup(-10...+10 V|0...20 mA|4...20 mA|0...10 V),popup(-10...+10 V|0...20 mA|4...20 mA|0...10 V),popup(FreeRun/SM-Synchron|DC-Synchron|DC-Synchron (input based)|DC-Customized),edit,checkbox,checkbox,edit,edit,edit,checkbox,edit,edit
      mask CallbackString: ||ep31xx('set');|||||ep31xx('set');||ep31xx('set');|||||||
      mask Display: fprintf('%s\nM:%i Idx:%s', model, master, mat2str(index));
  EP31xx_1 : S-Function  LoadFcn=|  FunctionName=ec_slave3  Parameters=Address,rv.SlaveConfig,rv.PortConfig,debug,tsample  SFunctionModules='ecrt_support'  EnableBusSupport=off  mask(EP31xx){master=0, index=1, model=EP3182-1002, revision=, type_1=-10...+10 V, type_2=-10...+10 V, type_3=-10...+10 V, type_4=-10...+10 V, filter=Off, vector=on, status=off, gain=[], offset=[], tau=[], tsample=0, debug=0, omega=, dc_mode=FreeRun/SM-Synchron, dc_assign_activate=hex2dec('700'), dc_cycle0=[], dc_cycle0_factor=[], dc_shift0=[], dc_shift0_factor=[], dc_shift0_input=off, dc_cycle1=[], dc_cycle1_factor=[], dc_shift1=[], dc_shift1_factor=[]}
      | ep31xx_1().checkModelName()
      | EtherCATSlave.checkFilter()
      mask prompts: index "Slave Index"; model "Device Model"; type_1 "Channel 1 Type"; type_2 "Channel 2 Type"; type_3 "Channel 3 Type"; type_4 "Channel 4 Type"; vector "Vector Ports"; status "Status Output"; gain "Output Scale (empty for none)"; offset "Output Offset (empty for none)"; tau "LPF time constant (s)"; tsample "Sample Time (-1 for inherited)"; omega "deprecated"; dc_mode "DC Mode"; dc_assign_activate "Assign Activate"; dc_cycle0 "Cycle Time Sync 0"; dc_cycle0_factor "Factor"; dc_shift0 "Shift Time Sync0"; dc_shift0_factor "Factor"; dc_shift0_input "Shift Time0 Input"; dc_cycle1 "Cycle Time Sync1"; dc_cycle1_factor "Factor"; dc_shift1 "Shift Time Sync1"; dc_shift1_factor "Factor"
      mask help: Beckhoff Analog Input 16-Bit Fieldbus Box
      mask init:
      | Address = EtherCATSlave.formatAddress(master,index,tsample);
      | 
      | rv = ep31xx_1(model).configure(status,vector,...
      |     EtherCATSlave.configureScale(2^15,gain,offset,tau),...
      |     [dc_mode, dc_assign_activate, ...
      |      dc_cycle0, dc_cycle0_factor, ...
      |      dc_shift0, dc_shift0_factor, dc_shift0_input, ...
      |      dc_cycle1, dc_cycle1_factor, ...
      |      dc_shift1, dc_shift1_factor], ...
      |      filter, [type_1,type_2,type_3,type_4]);
      |  
      | if isfield(rv.PortConfig,'input')
      |     inputnames = {rv.PortConfig.input.portname};
      | else
      |     inputnames = {};
      | end
      | 
      | if vector || model(6) == '1'
      |     set_param(gcb,'AttributesFormatString','');
      | 
      |     set_param(gcb,'MaskDisplay',...
      |         sprintf('disp(''%s\\nM:%i Idx:%s'')',...
      |         model,master,mat2str(index)))
      | else
      |     EtherCATSlave.setPortNames({},...
      |         {rv.PortConfig.output.portname})
      |     
      |     set_param(gcb,'AttributesFormatString',...
      |         sprintf('%s\nM:%i Idx:%s',...
      |         model,master,mat2str(index)))
      | end
      mask Help:
      | This block generically implements the EtherCAT 16-Bit Analog Input Fieldbus box Terminal for various models.
      | <p/>
      | The block input is generally a <tt>double</tt> from the range 0..1 for unipolar terminals and -1..1 for bipolar terminals, where 1 is the highest possible output of the terminal.
      | <p/>
      | Exceeding the input range simply saturates the terminal's output.
      | <p/>
      | The following Terminals are supported:
      | <center>
      | <table width="80%">
      | <tr><td>EP3174</td><td>4 port differential input</td></tr>
      | <tr><td>EP3182</td><td>2 port single ended input</td></tr>
      | <tr><td>EP3184</td><td>4 port single ended input</td></tr>
      | </table>
      | </center>
      | <p/>
      | Choose and set the following options:
      | <h4>Master:</h4>
      | Set the EtherCAT Master of this terminal.
      | 
      | <h4>Slave Index:</h4>
      | Set the EtherCAT slave index. Following address formats are allowed:
      | <ol>
      | <li> Absolute addressing: a scalar number <<b><tt>n</tt></b>> representing the (zero based) absolute position in the bus.
      | <li> SSId addressing: the Secondary Slave (or 'Alias') Addressing has the form <<b><tt>[alias position]</tt></b>> where <b><tt>alias</tt></b> is the Secondary Slave Id of the EtherCAT slave and <b><tt>position</tt></b> is the offset after the slave with the given <b><tt>alias</tt></b>. The SSId has to be preprogrammed into the slave with other service tools (see 'ethercat alias --help').
      | </ol>
      | 
      | <h4>Device Model:</h4>
      | Choose the device at the Indexed position of the master.
      | 
      | <h4>Channel 1-4 Type:</h4>
      | Choose the output type of the channel.
      | 
      | <h4>DC Mode:</h4>
      | Choose the DC Mode for the module.
      | 
      | <h4>DC Customer:</h4>
      | Do customized DC Settings in a vector
      | <<b><tt>[AssignActivate, CycleTimeSync0, CycleTimeSync0Factor, ShiftTimeSync0, ShiftTimeSync0Factor, ...
      | ShiftTimeSync0Input, CycleTimeSync1, CycleTimeSync1Factor, ShiftTimeSync1, ShiftTimeSync1Factor]</tt></b>>
      | 
      | <ul>
      | <li><<b><tt>AssignActivate:</tt></b>> Value for DC-mode setting
      | <li><<b><tt>CycleTimeSync0:</tt></b>> CycleTimeSync0 Value
      | <li><<b><tt>CycleTimeSync0Factor:</tt></b>> 1 or 0. If CycleTimeSync0Factor equals one the cycletimesync0 value is internally set to the process cycletime.
      | <li><<b><tt>ShiftTimeSync0:</tt></b>> ShiftTimeSync0 Value
      | <li><<b><tt>ShiftTimeSync0Factor:</tt></b>> 1 or 0. If ShiftTimeSync0Factor equals one the Slave is synced on the input event
      | <li><<b><tt>ShiftTimeSync0Input:</tt></b>> 1 or 0. If ShiftTimeSync0Input equals one the Slave is synced on the input event
      | <li><<b><tt>CycleTimeSync1:</tt></b>> CycleTimeSync1 Value
      | <li><<b><tt>CycleTimeSync1Factor:</tt></b>> 1 or 0. If CycleTimeSync1Factor equals one the CycletTimesSync1 value is internally set to the process cycletime.
      | <li><<b><tt>ShiftTimeSync1:</tt></b>>ShiftTimeSync1 Value
      | <li><<b><tt>ShiftTimeSync1Factor:</tt></b>> ShiftTimeSync1Factor Value
      | </ul>
      | 
      | <h4>Output Type:</h4>
      | <ul>
      | <li>Choose <b>Vector Output</b> to have a single output as a vector
      | with a size corresponding to the channel count of the terminal. This mode also allows a status output port to be displayed. <br/>
      | <li>Choose <b>Separate Outputs</b> to have one output for every channel.
      | </ul>
      | <h4>Output Full Scale</h4>
      | When <b>Output Data Type</b> is set to <b>Double with scale and offset</b>, the block's output value at full scale terminal input can be set here.
      | 
      | <h4>Output Offset</h4>
      | When <b>Output Data Type</b> is set to <b>Double with scale and offset</b>, the blocks output at zero terminal input can be set here. Note that the Full Scale above is also increased by this amount. Note furthermore that this corresponds to the minimum input for terminals such as 4..20mA.
      | 
      | <h4>Output Data Type</h4>
      | Choose the block's output data type for the output signal. Available are:
      | <ul>
      | <li><b><tt>Raw</tt></b> outputting the internal raw value as <tt>int16_T</tt> or <tt>uint16_T</tt> as appropriate
      | <li><b><tt>Double</tt></b> outputting 0..10, -10..10, 0..0.02 and 0.004..0.02 depending on the Model as appropriate
      | <li><b><tt>Double with scale and offset</tt></b>, allowing the output to be scaled with an offset.
      | </ul>
      | 
      | <p>
      | Choosing <b>Status Output</b> provides a port of type <tt>uint8_T</tt> where the status is presented. This is only enabled when <b>Vector Output</b> is selected. Terminal input over- and underrange can be detected using this output. See the terminal's documentation.
      | 
      | <h4>Output Filter</h4>
      | When not in <b>Raw</b> mode, the <b>Output Filter</b> checkbox becomes available, allowing the use of an internal low pass filter. Enter the <b>LPF Time Constant</b> for the filter in the field below.
      | <br>For continuous sample time systems (0 in Sample Time), the filter is also continuous. Discrete samples systems (Sample Time > 0) uses an equivalent discrete low pass filter with a similar time constant.
      | 
      | <p>
      | Set the <b>Sample Time</b> for the block. <tt>0</tt> is continuous sample time (runs at the model's base rate). Setting <tt>-1</tt> will try to set the time using back propagation.
      mask StyleString: edit,edit,popup(EP3174-0002|EP3182-1002|EP3184-0002|EP3184-1002),edit,popup(-10...+10 V|0...20 mA|4...20 mA|0...10 V),popup(-10...+10 V|0...20 mA|4...20 mA|0...10 V),popup(-10...+10 V|0...20 mA|4...20 mA|0...10 V),popup(-10...+10 V|0...20 mA|4...20 mA|0...10 V),popup(Off|50Hz FIR|60Hz FIR|IIR 1|IIR 2|IIR 3|IIR 4|IIR 5|IIR 6|IIR 7|IIR 8),checkbox,checkbox,edit,edit,edit,edit,edit,edit,popup(FreeRun/SM-Synchron|DC-Synchron|DC-Synchron (input based)|Custom),edit,min,max,min,max,checkbox,min,max,min,max
      mask CallbackString: ||ep31xx_1.modelChanged||||||ep31xx_1.updateFilter|||||||||EtherCATSlave.updateCustomDCEnable||||||||||
      mask TabNameString: Main,Main,Main,Main,Main,Main,Main,Main,Main,Main,Main,Main,Main,Main,Main,Main,Main,Distributed Clocks,Distributed Clocks,Distributed Clocks,Distributed Clocks,Distributed Clocks,Distributed Clocks,Distributed Clocks,Distributed Clocks,Distributed Clocks,Distributed Clocks,Distributed Clocks
      mask Display: disp('EP3182-1002\nM:0 Idx:1')
  EP41xx_0 : S-Function  LoadFcn=|  FunctionName=ec_slave3  Parameters=Address,rv.SlaveConfig,rv.PortConfig,debug,tsample  SFunctionModules='ecrt_support'  EnableBusSupport=off  mask(EP41xx){master=0, index=1, model=EP4174-0002, type_1=0...10 V, type_2=0...10 V, type_3=0...10 V, type_4=0...10 V, dcmode=FreeRun/SM-Synchron, dccustom=[hex2dec('730'),0,1,0,0,0,0,1,140000,0], vector=on, scale=, tsample=-1, debug=0}
      | ep41xx('check')
      | if ~strcmp(bdroot(gcb),'etherlab_lib')
      |   disp([gcb ' is obsolete. Please replace'])
      | end
      mask prompts: index "Slave Index"; model "Device Model"; type_1 "Channel 1 Type"; type_2 "Channel 2 Type"; type_3 "Channel 3 Type"; type_4 "Channel 4 Type"; dcmode "DC Mode"; dccustom "DC-Customized"; vector "Vector Input"; scale "Input Scale (empty for none)"; tsample "Sample Time (-1 for inherited)"
      mask help: Beckhoff Analog Output Fieldbus Box
      mask init:
      | Address = EtherCATSlave.formatAddress(master,index,tsample);
      | 
      | ep41xx('set');  % Report errors
      | 
      | rv = get_param(gcbh,'UserData');
      | 
      | basetype = [type_1; type_2; type_3; type_4] - 1;
      | type_eq3 = basetype == 3;
      | basetype = basetype .* ~type_eq3 + type_eq3*6;
      | 
      | rowcount = numel(rv.SlaveConfig.sm{1}{3});
      | 
      | rv.SlaveConfig.sdo = num2cell(horzcat(...
      |     hex2dec('F800')*ones(rowcount,1),...
      |     (1:rowcount)',...
      |     16*ones(rowcount,1),...
      |     basetype));
      mask Help:
      | This block generically implements the EtherCAT 16-Bit Analog Input Terminal for various fieldbus boxes.
      | <p/>
      | The block input is generally a <tt>double</tt> from the range 0..1 for unipolar terminals and -1..1 for bipolar terminals, where 1 is the highest possible output of the terminal.
      | <p/>
      | Exceeding the input range simply saturates the terminal's output.
      | <p/>
      | The following Terminals are supported:
      | <center>
      | <table width="80%">
      | <tr><td>EP4174</td><td>+/-10V, 0..10V,  Voltage Output or 0..20mA, 4..20mA Current Output</td></tr>
      | </table>
      | </center>
      | <p/>
      | Choose and set the following options:
      | <h4>Master:</h4>
      | Set the EtherCAT Master of this terminal.
      | 
      | <h4>Slave Index:</h4>
      | Set the EtherCAT slave index. Following address formats are allowed:
      | <ol>
      | <li> Absolute addressing: a scalar number <<b><tt>n</tt></b>> representing the (zero based) absolute position in the bus.
      | <li> SSId addressing: the Secondary Slave (or 'Alias') Addressing has the form <<b><tt>[alias position]</tt></b>> where <b><tt>alias</tt></b> is the Secondary Slave Id of the EtherCAT slave and <b><tt>position</tt></b> is the offset after the slave with the given <b><tt>alias</tt></b>. The SSId has to be preprogrammed into the slave with other service tools (see 'ethercat alias --help').
      | </ol>
      | 
      | <h4>Device Model:</h4>
      | Choose the device at the Indexed position of the master.
      | 
      | <h4>Channel 1-4 Type:</h4>
      | Choose the output type of the channel.
      | 
      | <h4>DC Mode:</h4>
      | Choose the DC Mode for the module.
      | 
      | <h4>DC Customized:</h4>
      | 
      | <<b><tt>[AssignActivate, CycleTimeSync0, CycleTimeSync0Factor, ShiftTimeSync0, ShiftTimeSync0Factor, ...
      | ShiftTimeSync0Input, CycleTimeSync1, CycleTimeSync1Factor, ShiftTimeSync1, ShiftTimeSync1Factor]</tt></b>>
      | 
      | <ul>
      | <li><<b><tt>AssignActivate:</tt></b>> Value for DC-mode setting
      | <li><<b><tt>CycleTimeSync0:</tt></b>> CycleTimeSync0 Value
      | <li><<b><tt>CycleTimeSync0Factor:</tt></b>> 1 or 0. If CycleTimeSync0Factor equals one the cycletimesync0 value is internally set to the process cycletime.
      | <li><<b><tt>ShiftTimeSync0:</tt></b>> ShiftTimeSync0 Value
      | <li><<b><tt>ShiftTimeSync0Factor:</tt></b>> 1 or 0. If ShiftTimeSync0Factor equals one the Slave is synced on the input event
      | <li><<b><tt>ShiftTimeSync0Input:</tt></b>> 1 or 0. If ShiftTimeSync0Input equals one the Slave is synced on the input event
      | <li><<b><tt>CycleTimeSync1:</tt></b>> CycleTimeSync1 Value
      | <li><<b><tt>CycleTimeSync1Factor:</tt></b>> 1 or 0. If CycleTimeSync1Factor equals one the CycletTimesSync1 value is internally set to the process cycletime.
      | <li><<b><tt>ShiftTimeSync1:</tt></b>>ShiftTimeSync1 Value
      | <li><<b><tt>ShiftTimeSync1Factor:</tt></b>> ShiftTimeSync1Factor Value
      | </ul>
      | 
      | <h4>Input Type:</h4>
      | <ul>
      | <li>Choose <b>Vector Input</b> to have a single input as a vector
      | with a size corresponding to the channel count of the terminal. This mode also allows a control input and a status output port to be displayed.
      | <li>Choose <b>Separate Inputs</b> to have one input for every channel.
      | </ul>
      | 
      | <p>
      | All input signals are multiplied with the factor <b>Input Scale</b>.
      | 
      | <p>
      | Set the <b>Sample Time</b> for the block. <tt>0</tt> is continuous sample time (runs at the model's base rate). Setting <tt>-1</tt> will try to set the time using back propagation.
      mask StyleString: edit,edit,popup(EP4174-0002),popup(-10...+10 V|0...20 mA|4...20 mA|0...10 V),popup(-10...+10 V|0...20 mA|4...20 mA|0...10 V),popup(-10...+10 V|0...20 mA|4...20 mA|0...10 V),popup(-10...+10 V|0...20 mA|4...20 mA|0...10 V),popup(FreeRun/SM-Synchron|DC-Synchron|DC-Customized),edit,checkbox,edit,edit,edit
      mask CallbackString: ||ep41xx('set')|||||ep41xx('set')||ep41xx('set')|||
      mask Display: fprintf('%s\nM:%i Idx:%s', model, master, mat2str(index))
  EP41xx_1 : S-Function  LoadFcn=ep41xx_1().checkModelName()  FunctionName=ec_slave3  Parameters=Address,rv.SlaveConfig,rv.PortConfig,debug,tsample  SFunctionModules='ecrt_support'  EnableBusSupport=off  mask(EP41xx){master=0, index=1, model=EP4174-0002, revision=, type_1=0...10 V, type_2=0...10 V, type_3=0...10 V, type_4=0...10 V, vector=on, gain=[], tsample=-1, debug=0, dc_mode=FreeRun/SM-Synchron, dc_assign_activate=hex2dec('730'), dc_cycle0=0, dc_cycle0_factor=1, dc_shift0=0, dc_shift0_factor=0, dc_shift0_input=off, dc_cycle1=0, dc_cycle1_factor=1, dc_shift1=140000, dc_shift1_factor=0}
      mask prompts: index "Slave Index"; model "Device Model"; type_1 "Channel 1 Type"; type_2 "Channel 2 Type"; type_3 "Channel 3 Type"; type_4 "Channel 4 Type"; vector "Vector Input"; gain "Input Scale (empty for none)"; tsample "Sample Time (-1 for inherited)"; dc_mode "DC Mode"; dc_assign_activate "Assign Activate"; dc_cycle0 "Cycle Time Sync 0"; dc_cycle0_factor "Factor"; dc_shift0 "Shift Time Sync0"; dc_shift0_factor "Factor"; dc_shift0_input "Shift Time0 Input"; dc_cycle1 "Cycle Time Sync1"; dc_cycle1_factor "Factor"; dc_shift1 "Shift Time Sync1"; dc_shift1_factor "Factor"
      mask help: Beckhoff Analog Output Fieldbus Box
      mask init:
      | Address = EtherCATSlave.formatAddress(master,index,tsample);
      | 
      | rv = ep41xx_1(model).configure(vector,...
      |     EtherCATSlave.configureScale(2^15,gain),...
      |     [dc_mode, dc_assign_activate, ...
      |      dc_cycle0, dc_cycle0_factor, ...
      |      dc_shift0, dc_shift0_factor, dc_shift0_input, ...
      |      dc_cycle1, dc_cycle1_factor, ...
      |      dc_shift1, dc_shift1_factor], ...
      |      [type_1; type_2; type_3; type_4]);
      mask Help:
      | This block generically implements the EtherCAT 16-Bit Analog Input Terminal for various fieldbus boxes.
      | <p/>
      | The block input is generally a <tt>double</tt> from the range 0..1 for unipolar terminals and -1..1 for bipolar terminals, where 1 is the highest possible output of the terminal.
      | <p/>
      | Exceeding the input range simply saturates the terminal's output.
      | <p/>
      | The following Terminals are supported:
      | <center>
      | <table width="80%">
      | <tr><td>EP4174</td><td>+/-10V, 0..10V,  Voltage Output or 0..20mA, 4..20mA Current Output</td></tr>
      | </table>
      | </center>
      | <p/>
      | Choose and set the following options:
      | <h4>Master:</h4>
      | Set the EtherCAT Master of this terminal.
      | 
      | <h4>Slave Index:</h4>
      | Set the EtherCAT slave index. Following address formats are allowed:
      | <ol>
      | <li> Absolute addressing: a scalar number <<b><tt>n</tt></b>> representing the (zero based) absolute position in the bus.
      | <li> SSId addressing: the Secondary Slave (or 'Alias') Addressing has the form <<b><tt>[alias position]</tt></b>> where <b><tt>alias</tt></b> is the Secondary Slave Id of the EtherCAT slave and <b><tt>position</tt></b> is the offset after the slave with the given <b><tt>alias</tt></b>. The SSId has to be preprogrammed into the slave with other service tools (see 'ethercat alias --help').
      | </ol>
      | 
      | <h4>Device Model:</h4>
      | Choose the device at the Indexed position of the master.
      | 
      | <h4>Channel 1-4 Type:</h4>
      | Choose the output type of the channel.
      | 
      | <h4>DC Mode:</h4>
      | Choose the DC Mode for the module.
      | 
      | <h4>DC Customized:</h4>
      | 
      | <<b><tt>[AssignActivate, CycleTimeSync0, CycleTimeSync0Factor, ShiftTimeSync0, ShiftTimeSync0Factor, ...
      | ShiftTimeSync0Input, CycleTimeSync1, CycleTimeSync1Factor, ShiftTimeSync1, ShiftTimeSync1Factor]</tt></b>>
      | 
      | <ul>
      | <li><<b><tt>AssignActivate:</tt></b>> Value for DC-mode setting
      | <li><<b><tt>CycleTimeSync0:</tt></b>> CycleTimeSync0 Value
      | <li><<b><tt>CycleTimeSync0Factor:</tt></b>> 1 or 0. If CycleTimeSync0Factor equals one the cycletimesync0 value is internally set to the process cycletime.
      | <li><<b><tt>ShiftTimeSync0:</tt></b>> ShiftTimeSync0 Value
      | <li><<b><tt>ShiftTimeSync0Factor:</tt></b>> 1 or 0. If ShiftTimeSync0Factor equals one the Slave is synced on the input event
      | <li><<b><tt>ShiftTimeSync0Input:</tt></b>> 1 or 0. If ShiftTimeSync0Input equals one the Slave is synced on the input event
      | <li><<b><tt>CycleTimeSync1:</tt></b>> CycleTimeSync1 Value
      | <li><<b><tt>CycleTimeSync1Factor:</tt></b>> 1 or 0. If CycleTimeSync1Factor equals one the CycletTimesSync1 value is internally set to the process cycletime.
      | <li><<b><tt>ShiftTimeSync1:</tt></b>>ShiftTimeSync1 Value
      | <li><<b><tt>ShiftTimeSync1Factor:</tt></b>> ShiftTimeSync1Factor Value
      | </ul>
      | 
      | <h4>Input Type:</h4>
      | <ul>
      | <li>Choose <b>Vector Input</b> to have a single input as a vector
      | with a size corresponding to the channel count of the terminal. This mode also allows a control input and a status output port to be displayed.
      | <li>Choose <b>Separate Inputs</b> to have one input for every channel.
      | </ul>
      | 
      | <p>
      | All input signals are multiplied with the factor <b>Input Scale</b>.
      | 
      | <p>
      | Set the <b>Sample Time</b> for the block. <tt>0</tt> is continuous sample time (runs at the model's base rate). Setting <tt>-1</tt> will try to set the time using back propagation.
      mask StyleString: edit,edit,popup(EP4174-0002),edit,popup(-10...+10 V|0...20 mA|4...20 mA|0...10 V),popup(-10...+10 V|0...20 mA|4...20 mA|0...10 V),popup(-10...+10 V|0...20 mA|4...20 mA|0...10 V),popup(-10...+10 V|0...20 mA|4...20 mA|0...10 V),checkbox,edit,edit,edit,popup(FreeRun/SM-Synchron|DC-Synchron|Custom),edit,min,max,min,max,checkbox,min,max,min,max
      mask CallbackString: ||ep41xx_1().updateRevision()||||||||||EtherCATSlave.updateCustomDCEnable()||||||||||
      mask TabNameString: Main,Main,Main,Main,Main,Main,Main,Main,Main,Main,Main,Main,Distributed Clocks,Distributed Clocks,Distributed Clocks,Distributed Clocks,Distributed Clocks,Distributed Clocks,Distributed Clocks,Distributed Clocks,Distributed Clocks,Distributed Clocks,Distributed Clocks
      mask Display: fprintf('%s\nM:%i Idx:%s', model, master, mat2str(index))
  EP43xx_0 : S-Function  LoadFcn=|  FunctionName=ec_slave3  Parameters=Address,rv.SlaveConfig,rv.PortConfig,debug,tsample  SFunctionModules='ecrt_support'  EnableBusSupport=off  mask(EP4374){master=0, index=1, model=EP4374-0002, type_1=0...10 V, type_2=0...10 V, type_3=0...10 V, type_4=0...10 V, status=off, vector=on, dcmode=FreeRun/SM-Synchron, dccustom=[hex2dec('700') 0 1 0 0 0 0 1 80000 0], i_scale=[], o_scale=[], o_offset=[], tau=[], force=off, tsample=0, debug=0}
      | ep43xx('check');
      | if ~strcmp(bdroot(gcb),'etherlab_lib')
      |   disp([gcb ' is obsolete. Please replace'])
      | end
      mask prompts: index "Slave Index"; model "Device Model"; type_1 "Input type Ch1"; type_2 "Input type Ch2"; type_3 "Output type Ch3"; type_4 "Output type Ch4"; status "Status Output"; vector "Vector IO"; dcmode "DC Mode"; dccustom "DC Customer"; i_scale "Input Scale"; o_scale "Output Scale"; o_offset "Output Offset"; tau "LPF Time Constant (sec)"; force "IO Force"; tsample "Sample Time (-1 for inherited)"
      mask help: Beckhoff Analog Input/Output 16-Bit Fieldbus Box
      mask init:
      | Address = EtherCATSlave.formatAddress(master,index,tsample);
      | 
      | ep43xx('set');
      | 
      | rv = get_param(gcbh,'UserData');
      | 
      | rowcount = numel(rv.SlaveConfig.sm{1}{3}) ...
      |          + numel(rv.SlaveConfig.sm{2}{3});
      | 
      | rv.SlaveConfig.sdo = num2cell(horzcat(...
      |     hex2dec('F800')*ones(rowcount,1),...
      |     (1:rowcount)',...
      |     16*ones(rowcount,1),...
      |     [type_1; type_2; type_3; type_4] - 1));
      mask Help: web(etherlab_help_path('ep43xx.html'), '-helpbrowser')
      mask StyleString: edit,edit,popup(EP4374-0002),popup(-10...+10 V|0...20 mA|4...20 mA|0...10 V),popup(-10...+10 V|0...20 mA|4...20 mA|0...10 V),popup(-10...+10 V|0...20 mA|4...20 mA|0...10 V),popup(-10...+10 V|0...20 mA|4...20 mA|0...10 V),checkbox,checkbox,popup(FreeRun/SM-Synchron|DC-Synchron|DC-Customized),edit,edit,edit,edit,edit,checkbox,edit,edit
      mask CallbackString: ||ep43xx('set');|||||ep43xx('set');|ep43xx('set');|ep43xx('ui');||||||||
      mask Display: fprintf('%s\nAnalog IO\nM:%i Idx:%s', model, master, mat2str(index));
  EP43xx_1 : S-Function  LoadFcn=|  FunctionName=ec_slave3  Parameters=Address,rv.SlaveConfig,rv.PortConfig,debug,tsample  SFunctionModules='ecrt_support'  EnableBusSupport=off  mask(EP4374){master=0, index=1, model=EP4374-0002, revision=, vector=on, tsample=-1, debug=0, type_1=0...10 V, type_2=-10...+10 V, filter=Off, status=off, o_gain=[], o_offset=[], tau=[], omega=, type_3=-10...+10 V, type_4=-10...+10 V, i_gain=[], dc_mode=FreeRun/SM-Synchron, dc_assign_activate=hex2dec('700'), dc_cycle0=[], dc_cycle0_factor=[], dc_shift0=[], dc_shift0_factor=[], dc_shift0_input=off, dc_cycle1=[], dc_cycle1_factor=[], dc_shift1=[], dc_shift1_factor=[]}
      | ep43xx_1().checkModelName()
      | EtherCATSlave.checkFilter()
      mask prompts: index "Slave Index"; model "Device Model"; vector "Vector IO"; tsample "Sample Time (-1 for inherited)"; type_1 "Analog Input type Ch1"; type_2 "Analog Input type Ch2"; o_gain "Scale"; o_offset "Offset"; tau "LPF time constant (s)"; omega "deprecated"; type_3 "Analog Output type Ch3"; type_4 "Analog Output type Ch4"; i_gain "Scale"; dc_mode "DC Mode"; dc_assign_activate "Assign Activate"; dc_cycle0 "Cycle Time Sync 0"; dc_cycle0_factor "Factor"; dc_shift0 "Shift Time Sync0"; dc_shift0_factor "Factor"; dc_shift0_input "Shift Time0 Input"; dc_cycle1 "Cycle Time Sync1"; dc_cycle1_factor "Factor"; dc_shift1 "Shift Time Sync1"; dc_shift1_factor "Factor"
      mask help: Beckhoff Analog Input/Output 16-Bit Fieldbus Box
      mask init:
      | Address = EtherCATSlave.formatAddress(master,index,tsample);
      | 
      | rv = ep43xx_1(model).configure(status,vector,...
      |     EtherCATSlave.configureScale(2^15,o_gain,o_offset,tau,'I'),...
      |     EtherCATSlave.configureScale(2^15,i_gain,[],[],'O'),...
      |     [dc_mode, dc_assign_activate, ...
      |      dc_cycle0, dc_cycle0_factor, ...
      |      dc_shift0, dc_shift0_factor, dc_shift0_input, ...
      |      dc_cycle1, dc_cycle1_factor, ...
      |      dc_shift1, dc_shift1_factor],...
      |      filter,[type_1,type_2,type_3,type_4]);
      mask Help: web(etherlab_help_path('ep43xx.html'), '-helpbrowser')
      mask StyleString: edit,edit,popup(EP4374-0002),edit,checkbox,edit,edit,popup(-10...+10 V|0...20 mA|4...20 mA|0...10 V),popup(-10...+10 V|0...20 mA|4...20 mA|0...10 V),popup(Off|50Hz FIR|60Hz FIR|IIR 1|IIR 2|IIR 3|IIR 4|IIR 5|IIR 6|IIR 7|IIR 8),checkbox,edit,edit,edit,edit,popup(-10...+10 V|0...20 mA|4...20 mA|0...10 V),popup(-10...+10 V|0...20 mA|4...20 mA|0...10 V),edit,popup(FreeRun/SM-Synchron|DC-Synchron|Custom),edit,min,max,min,max,checkbox,min,max,min,max
      mask CallbackString: ||ep43xx_1().updateRevision||||||||||||||||EtherCATSlave.updateCustomDCEnable()||||||||||
      mask TabNameString: Main,Main,Main,Main,Main,Main,Main,Input,Input,Input,Input,Input,Input,Input,Input,Output,Output,Output,Distributed Clocks,Distributed Clocks,Distributed Clocks,Distributed Clocks,Distributed Clocks,Distributed Clocks,Distributed Clocks,Distributed Clocks,Distributed Clocks,Distributed Clocks,Distributed Clocks
      mask Display: fprintf('%s\nAnalog IO\nM:%iIdx:%s', model, master, mat2str(index));
  EP8309_0 : S-Function  LoadFcn=ep8309().checkModelName()  FunctionName=ec_slave3  Parameters=Address,rv.SlaveConfig,rv.PortConfig,debug,tsample  SFunctionModules='ecrt_support'  EnableBusSupport=off  mask(EP8309){master=0, index=1, model=EP8309-1022, revision=, tsample=0, debug=0, digin=on, digout=on, devstat=off, anain=off, gain=[], offset=[], tau=[], sdo_F800_01=0..20 mA, sdo_F800_02=0..20 mA, sdo_8000_15=Off, filter=, tacho=None, sdo_8020_11=1, sdo_8020_12=100, sdo_8020_15=RPM, sdo_8030_11=1, sdo_8030_12=100, sdo_8030_15=RPM, sdo_8031_0B=on, sdo_8031_0C=off, sdo_8031_11=1, sdo_8031_12=100, sdo_8031_15=RPM, anaout=None, gain2=[], sdo_8050_03=off, sdo_8050_04=off, sdo_8050_05=Set to default, sdo_8050_0D=0, sdo_8050_0E=65535, sdo_8050_10=100, sdo_8050_12=250, sdo_8050_13=4, sdo_8050_14=50, sdo_8050_1E=64, sdo_8050_1F=10, sdo_8060_05=Set to default, sdo_8060_13=4, sdo_8060_14=50, sdo_F800_08=0..20 mA}
      mask prompts: index "Slave Index"; model "Device Model"; tsample "Sample Time (-1 inherited)"; digin "Digital Input"; digout "Digital Output"; devstat "Device Status"; anain "Analog Input"; tau "LPF time constant (s)"; sdo_F800_01 "F800:01 - Output type Ch.1"; sdo_F800_02 "F800:02 - Output type Ch.2"; sdo_8000_15 "8000:06/15 - Hardware filter"; filter "deprecated"; tacho "Tacho Input"; sdo_8020_11 "8020:11 - Targets 1"; sdo_8020_12 "8020:12 - Timeout 1"; sdo_8020_15 "8020:15 - Presentation 1"; sdo_8030_11 "8030:11 - Targets 2"; sdo_8030_12 "8030:12 - Timeout 2"; sdo_8030_15 "8030:15 - Presentation 2"; sdo_8031_0B "8031:0B - Error detection"; sdo_8031_0C "8031:0C - Reversion of rotation"; sdo_8031_11 "8031:11 - Targets"; sdo_8031_12 "8031:12 - Timeout"; sdo_8031_15 "8031:15 - Presentation"; anaout "Analog Output"; gain2 "Gain"; sdo_8050_03 "8050:03 - Dithering"; sdo_8050_04 "8050:04 - Invert polarity"; sdo_8050_05 "8050:05 - Watchdog"; sdo_8050_0D "8050:0D - Default output"; sdo_8050_0E "8050:0E - Default output ramp"; sdo_8050_10 "8050:10 - Max Current [%]"; sdo_8050_12 "8050:12 - Kp factor"; sdo_8050_13 "8050:13 - Ki factor"; sdo_8050_14 "8050:14 - Kd factor"; sdo_8050_1E "8050:1E - Dither frequency [Hz]"; sdo_8050_1F "8050:1F - Dither amplitude [%]"; sdo_8060_05 "8060:05 - Watchdog"; sdo_8060_13 "8060:13 - Default output"; sdo_8060_14 "8060:14 - Default output ramp"; sdo_F800_08 "F800:08 - Output type"
      mask help: Beckhoff Multifunctional I/O EtherCAT Box
      mask init:
      | Address = EtherCATSlave.formatAddress(master,index,tsample);
      | 
      | io = [];
      | 
      | if digin
      |     io.digin = 1;
      | end
      | if digout
      |     io.digout = 1;
      | end
      | if devstat
      |     io.devstat = 1;
      | end
      | if anain
      |     io.anain.gain = gain;
      |     io.anain.offset = offset;
      |     io.anain.filter = tau;
      |     io.anain.sdo = [hex2dec('8000'), hex2dec('06'), sdo_8000_15 > 1;
      |                     hex2dec('8000'), hex2dec('15'), sdo_8000_15 - 1;
      |                     hex2dec('F800'), hex2dec('01'), sdo_F800_01;
      |                     hex2dec('F800'), hex2dec('02'), sdo_F800_02];
      | end
      | tachogain = [1,0.1,0.01,1,0.1,0.01,0.001];
      | switch tacho
      |     case 2  % Single shaft mode
      |         io.tacho1.gain = tachogain(sdo_8031_15);
      |         io.tacho1.sdo = [hex2dec('8031'), hex2dec('0B'), sdo_8031_0B;
      |                          hex2dec('8031'), hex2dec('0C'), sdo_8031_0C;
      |                          hex2dec('8031'), hex2dec('11'), sdo_8031_11;
      |                          hex2dec('8031'), hex2dec('12'), sdo_8031_12;
      |                          hex2dec('8031'), hex2dec('15'), sdo_8031_15];
      |     case 3   % dual shaft mode
      |         io.tacho2.gain = [tachogain(sdo_8020_15), tachogain(sdo_8030_15)];
      |         io.tacho2.sdo = [hex2dec('8020'), hex2dec('11'), sdo_8020_11;
      |                          hex2dec('8020'), hex2dec('12'), sdo_8020_12;
      |                          hex2dec('8020'), hex2dec('15'), sdo_8020_15;
      |                          hex2dec('8030'), hex2dec('11'), sdo_8030_11;
      |                          hex2dec('8030'), hex2dec('12'), sdo_8030_12;
      |                          hex2dec('8030'), hex2dec('15'), sdo_8030_15];
      | end
      | switch anaout
      |     case 2  % Current
      |         io.current.gain = gain2;
      |         io.current.sdo = [hex2dec('8060'), hex2dec('05'), sdo_8060_05;
      |                           hex2dec('8060'), hex2dec('13'), sdo_8060_13;
      |                           hex2dec('8060'), hex2dec('14'), sdo_8060_14;
      |                           hex2dec('F800'), hex2dec('08'), sdo_F800_08];
      |     case 3  % PWM
      |         io.pwm.gain = gain2;
      |         io.pwm.sdo = [hex2dec('8050'), hex2dec('03'), sdo_8050_03;
      |                       hex2dec('8050'), hex2dec('04'), sdo_8050_04;
      |                       hex2dec('8050'), hex2dec('05'), sdo_8050_05;
      |                       hex2dec('8050'), hex2dec('0D'), sdo_8050_0D;
      |                       hex2dec('8050'), hex2dec('0E'), sdo_8050_0E;
      |                       hex2dec('8050'), hex2dec('10'), sdo_8050_10;
      |                       hex2dec('8050'), hex2dec('12'), sdo_8050_12;
      |                       hex2dec('8050'), hex2dec('13'), sdo_8050_13;
      |                       hex2dec('8050'), hex2dec('14'), sdo_8050_14;
      |                       hex2dec('8050'), hex2dec('1E'), sdo_8050_1E;
      |                       hex2dec('8050'), hex2dec('1F'), sdo_8050_1F];
      | end
      | 
      | %save ep
      | rv = ep8309(model).configure(io);
      | 
      | EtherCATSlave.setPortNames(...
      |     {rv.PortConfig.input.portname},...
      |     {rv.PortConfig.output.portname});
      | 
      | set_param(gcb,'AttributesFormatString',...
